simulink model "Centralized_Cont"  (R2018a)
settings: Solver=VariableStepAuto  StartTime=0.0  StopTime=5  RelTol=1e-3
values from neighbouring files (symbols this model uses):
  Kd_Cent = zeros(7,7)    [ControlSetup.m]
  Kp_Cent = zeros(7,7)    [ControlSetup.m]
libraries: dspinverses x1
(part 4 of 4)

== matlab function Centralized_Cont/Estimator/Dynamics_e ==
  data: dq2 input; B output; dq3 input; dq4 input; dq5 input; dq6 input; dq7 input; g input; q2 input; q3 input; q4 input; q5 input; q6 input; Bm output; phi output; phim output; G output
function [B,Bm,phi,phim,G] = Dynamics_e(dq2,dq3,dq4,dq5,dq6,dq7,g,q2,q3,q4,q5,q6)
%#codegen

%    This function was generated by the Symbolic Math Toolbox version 8.1.
%    29-May-2020 11:22:38

t2 = cos(q2);
t3 = sin(q2);
t4 = sin(q5);
t5 = cos(q3);
t6 = cos(q4);
t7 = sin(q3);
t8 = sin(q4);
t9 = cos(q5);
t10 = cos(q6);
t11 = sin(q6);
t12 = t3.*4.525398e-2;
t13 = t3.*t4.*t11.*1.279539e-2;
t14 = t2.*t5.*t8.*1.27482732;
t15 = t2.*t6.*t7.*1.27482732;
t16 = t2.*t7.*t8.*2.136096e-1;
t17 = t2.*t4.*t5.*t6.*1.612305e-2;
t18 = t2.*t5.*t8.*t10.*1.279539e-2;
t19 = t2.*t6.*t7.*t10.*1.279539e-2;
t20 = t2.*t7.*t8.*t9.*4.1238e-4;
t21 = t2.*t5.*t6.*t9.*t11.*1.279539e-2;
t22 = t2.*(-5.811597e-1)+t12+t13+t14+t15+t16+t17+t18+t19+t20+t21-t2.*t5.*4.3309791-t3.*t4.*4.1238e-4-t2.*t7.*5.866623e-2-t3.*t9.*1.612305e-2-t2.*t5.*t6.*2.136096e-1-t2.*t4.*t7.*t8.*1.612305e-2-t2.*t5.*t6.*t9.*4.1238e-4-t2.*t7.*t8.*t9.*t11.*1.279539e-2;
t23 = t5.^2;
t24 = t6.^2;
t25 = t10.^2;
t26 = t9.^2;
t27 = t5.*t8.*1.484568e-6;
t28 = t6.*t7.*1.484568e-6;
t29 = t4.*t7.*t8.*9.5218542e-5;
t30 = t7.*t8.*t9.*4.194107562e-3;
t31 = t5.*t8.*t11.*t26.*4.2919632e-5;
t32 = t6.*t7.*t11.*t26.*4.2919632e-5;
t33 = t4.*t5.*t8.*t9.*2.159275886e-3;
t34 = t4.*t6.*t7.*t9.*2.159275886e-3;
t35 = t4.*t5.*t6.*t11.*4.67031735e-3;
t36 = t7.*t8.*t9.*t10.*2.1459816e-5;
t37 = t4.*t5.*t8.*t11.*4.4783865e-4;
t38 = t4.*t6.*t7.*t11.*4.4783865e-4;
t39 = t4.*t5.*t8.*t9.*t25.*7.96554327e-4;
t40 = t4.*t6.*t7.*t9.*t25.*7.96554327e-4;
t41 = t4.*t5.*t6.*t10.*t11.*7.96554327e-4;
t42 = t5.*6.880448217896662e19;
t43 = t7.*5.079426005445158e21;
t44 = t7.*t8.*1.495133292529617e21;
t45 = t4.*t5.*t8.*1.890931301356143e19;
t46 = t4.*t6.*t7.*1.890931301356143e19;
t47 = t7.*t8.*t10.*1.5006592092724e19;
t48 = t5.*t8.*t9.*t11.*1.5006592092724e19;
t49 = t6.*t7.*t9.*t11.*1.5006592092724e19;
t50 = t42-t43+t44+t45+t46+t47+t48+t49-t5.*t6.*1.495133292529617e21-t5.*t8.*2.505239882715523e20-t6.*t7.*2.505239882715523e20-t5.*t6.*t10.*1.5006592092724e19-t5.*t8.*t9.*4.836443787330847e17-t6.*t7.*t9.*4.836443787330847e17;
t51 = t7.*1.121030218e-2;
t52 = t4.*t7.*t11.*4.03054785e-3;
t68 = t5.*t8.*t26.*2.969136e-6;
t69 = t6.*t7.*t26.*2.969136e-6;
t70 = t5.*t6.*t9.*4.194107562e-3;
t71 = t4.*t5.*t6.*9.5218542e-5;
t72 = t5.*t8.*t9.*5.6430675e-4;
t73 = t6.*t7.*t9.*5.6430675e-4;
t74 = t4.*t5.*t8.*1.44333e-5;
t75 = t4.*t6.*t7.*1.44333e-5;
t76 = t5.*t8.*t11.*2.1459816e-5;
t77 = t6.*t7.*t11.*2.1459816e-5;
t78 = t5.*t6.*t9.*t10.*2.1459816e-5;
t79 = t4.*t7.*t8.*t11.*4.67031735e-3;
t80 = t4.*t7.*t8.*t10.*t11.*7.96554327e-4;
t53 = t5.*(-3.40264134e-4)+t27+t28+t29+t30+t31+t32+t33+t34+t35+t36+t37+t38+t39+t40+t41+t51+t52-t68-t69-t70-t71-t72-t73-t74-t75-t76-t77-t78-t79-t80-t4.*t7.*1.298997e-4-t7.*t9.*5.07876075e-3;
t54 = t9.*2.88666e-5;
t55 = q5.*2.0;
t56 = sin(t55);
t57 = t10.*9.3406347e-3;
t58 = t25.*7.96554327e-4;
t59 = t4.*t9.*t11.*4.2919632e-5;
t60 = t5.*t6.*1.4164748e7;
t61 = t5.*t8.*2.37344e6;
t62 = t6.*t7.*2.37344e6;
t63 = t5.*t6.*t10.*1.42171e5;
t64 = t5.*t8.*t9.*4.582e3;
t65 = t6.*t7.*t9.*4.582e3;
t66 = t60+t61+t62+t63+t64+t65-t7.*t8.*1.4164748e7-t4.*t5.*t8.*1.79145e5-t4.*t6.*t7.*1.79145e5-t7.*t8.*t10.*1.42171e5-t5.*t8.*t9.*t11.*1.42171e5-t6.*t7.*t9.*t11.*1.42171e5;
t67 = t3.*t66.*9.0e-8;
t81 = t6.*6.7287024e-2;
t82 = t6.*t9.*1.298997e-4;
t84 = t56.*1.484568e-6;
t85 = t4.*1.1286135e-3;
t86 = t9.*t11.*8.956773e-4;
t87 = t26.*2.159275886e-3;
t88 = t25.*t26.*7.96554327e-4;
t83 = t8.*(-4.015706058e-1)+t54+t57+t58+t59+t81+t82-t84-t85-t86-t87-t88-t4.*t6.*5.07876075e-3-t8.*t10.*4.03054785e-3-t6.*t9.*t11.*4.03054785e-3+3.67536334659e-1;
t89 = t9.*4.194107562e-3;
t90 = t4.*9.5218542e-5;
t91 = t9.*t10.*2.1459816e-5;
t92 = t9.*1.201554327e-3;
t93 = t9.*t10.*4.67031735e-3;
t94 = t4.*t11.*2.1459816e-5;
t95 = t4.*t11.*5.0e-6;
t96 = t2.*t9.*4.1238e-4;
t97 = t3.*t5.*t6.*t9.*1.612305e-2;
t98 = t3.*t4.*t5.*t6.*4.1238e-4;
t99 = t3.*t4.*t7.*t8.*t11.*1.279539e-2;
t100 = t96+t97+t98+t99-t2.*t4.*1.612305e-2-t2.*t9.*t11.*1.279539e-2-t3.*t4.*t7.*t8.*4.1238e-4-t3.*t7.*t8.*t9.*1.612305e-2-t3.*t4.*t5.*t6.*t11.*1.279539e-2;
t101 = t4.*4.0307625e-4;
t102 = t4.*t5.*5.07876075e-3;
t103 = t9.*t11.*3.1988475e-4;
t104 = t7.*t8.*1.0957467016e-2;
t105 = t5.*t6.*t25.*7.96554327e-4;
t106 = t4.*t5.*t6.*5.6430675e-4;
t107 = t5.*t8.*t9.*9.5218542e-5;
t108 = t6.*t7.*t9.*9.5218542e-5;
t109 = t5.*t9.*t11.*4.03054785e-3;
t110 = t7.*t8.*t9.*1.44333e-5;
t111 = t5.*t6.*t9.*t11.*4.4783865e-4;
t112 = t9.*(-1.03095e-5)+t101+t102+t103+t104+t105+t106+t107+t108+t109+t110+t111-t5.*t6.*1.0957467016e-2-t5.*t9.*1.298997e-4-t4.*t5.*t8.*4.194107562e-3-t4.*t6.*t7.*4.194107562e-3-t4.*t7.*t8.*5.6430675e-4-t5.*t6.*t9.*1.44333e-5-t7.*t8.*t25.*7.96554327e-4-t4.*t5.*t8.*t10.*2.1459816e-5-t4.*t6.*t7.*t10.*2.1459816e-5-t5.*t8.*t9.*t11.*4.67031735e-3-t6.*t7.*t9.*t11.*4.67031735e-3-t7.*t8.*t9.*t11.*4.4783865e-4-t5.*t8.*t9.*t10.*t11.*7.96554327e-4-t6.*t7.*t9.*t10.*t11.*7.96554327e-4;
t113 = t4.*t8.*t11.*4.03054785e-3;
t115 = t4.*t11.*4.67031735e-3;
t116 = t4.*t10.*t11.*7.96554327e-4;
t114 = t89+t90+t91+t113-t115-t116-t4.*t8.*1.298997e-4-t8.*t9.*5.07876075e-3;
t117 = t3.*t5.*t6.*t9.*t10.*1.279539e-2;
t118 = t117-t2.*t4.*t10.*1.279539e-2-t3.*t5.*t8.*t11.*1.279539e-2-t3.*t6.*t7.*t11.*1.279539e-2-t3.*t7.*t8.*t9.*t10.*1.279539e-2;
t119 = t4.*t10.*3.1988475e-4;
t120 = t4.*t5.*t10.*4.03054785e-3;
t121 = t7.*t8.*t10.*2.1459816e-5;
t122 = t4.*t5.*t6.*t10.*4.4783865e-4;
t123 = t5.*t8.*t9.*t11.*2.1459816e-5;
t124 = t6.*t7.*t9.*t11.*2.1459816e-5;
t125 = t119+t120+t121+t122+t123+t124-t4.*t5.*t8.*1.201554327e-3-t4.*t6.*t7.*1.201554327e-3-t5.*t6.*t10.*2.1459816e-5-t4.*t5.*t8.*t10.*4.67031735e-3-t4.*t6.*t7.*t10.*4.67031735e-3-t4.*t7.*t8.*t10.*4.4783865e-4;
t127 = t11.*4.4783865e-4;
t126 = t92+t93+t94-t127-t6.*t11.*4.03054785e-3-t8.*t9.*t10.*4.03054785e-3;
t128 = t10.*2.1459816e-5;
t129 = q3+q4;
t130 = t10.*5.0e-6;
t131 = q4.*2.0;
t132 = t11.^2;
t133 = t4.*t10.*(2.1e1./1.0e3);
t134 = t9.*t10.*t11.*(2.1e1./1.0e3);
t135 = t133+t134;
t136 = t4.^2;
t140 = t4.*t11;
t137 = t9-t140;
t138 = sin(t129);
t139 = cos(t129);
t141 = dq2.^2;
t142 = dq5.^2;
t143 = dq3.^2;
t144 = dq4.^2;
t145 = dq6.^2;
t146 = q3.*2.0;
t147 = sin(t146);
t148 = cos(t55);
t149 = cos(t146);
t150 = cos(t131);
t151 = sin(t131);
B = reshape([7.8426e1,t22,t3.*t50.*(-8.526512829121202e-22),t67,t100,t118,0.0,t22,t4.*(-1.1286135e-3)+t5.*2.16548955e-1+t7.*2.9333115e-3+t23.*1.610619881558+t24.*3.25881982477e-1-t25.*7.96554327e-4+t54+t147.*5.438968859e-2+t151.*4.520441246e-2+t5.*t6.*1.068048e-2-t5.*t8.*6.3741366e-2-t6.*t7.*6.3741366e-2-t7.*t8.*1.068048e-2-t9.*t11.*8.956773e-4+t4.*t23.*1.1286135e-3+t4.*t24.*1.1286135e-3+t6.*t23.*1.34574048e-1-t8.*t23.*8.031412116e-1-t9.*t23.*2.88666e-5-t9.*t24.*2.88666e-5+t10.*t23.*9.3406347e-3+t10.*t24.*9.3406347e-3-t23.*t24.*6.51763964954e-1+t23.*t25.*7.96554327e-4+t23.*t26.*2.159275886e-3+t24.*t25.*7.96554327e-4+t24.*t26.*2.159275886e-3-t4.*t5.*t6.*8.061525e-4-t4.*t5.*t7.*8.388215124e-3-t4.*t6.*t8.*8.388215124e-3-t5.*t6.*t7.*8.031412116e-1+t4.*t7.*t8.*8.061525e-4+t5.*t6.*t9.*2.0619e-5-t5.*t7.*t8.*1.34574048e-1+t5.*t7.*t9.*1.90437084e-4+t5.*t7.*t10.*8.956773e-4-t5.*t8.*t10.*6.397695e-4-t6.*t7.*t10.*6.397695e-4+t6.*t8.*t9.*1.90437084e-4+t6.*t8.*t10.*8.956773e-4-t7.*t8.*t9.*2.0619e-5-t4.*t6.*t23.*1.01575215e-2+t4.*t9.*t23.*2.969136e-6-t5.*t7.*t24.*1.8081764984e-1+t4.*t9.*t24.*2.969136e-6-t6.*t8.*t23.*1.8081764984e-1+t6.*t9.*t23.*2.597994e-4-t8.*t10.*t23.*8.0610957e-3+t9.*t11.*t23.*8.956773e-4+t9.*t11.*t24.*8.956773e-4-t4.*t23.*t24.*2.257227e-3+t9.*t23.*t24.*5.77332e-5-t10.*t23.*t24.*1.86812694e-2-t23.*t24.*t25.*1.593108654e-3-t23.*t24.*t26.*4.318551772e-3+t23.*t25.*t26.*7.96554327e-4+t24.*t25.*t26.*7.96554327e-4+t4.*t5.*t7.*t8.*1.01575215e-2-t4.*t5.*t7.*t10.*4.2919632e-5+t5.*t6.*t7.*t8.*6.51763964954e-1-t4.*t6.*t8.*t10.*4.2919632e-5-t5.*t6.*t7.*t10.*8.0610957e-3-t5.*t7.*t8.*t9.*2.597994e-4-t5.*t6.*t9.*t11.*6.397695e-4-t5.*t7.*t9.*t11.*9.3406347e-3-t6.*t8.*t9.*t11.*9.3406347e-3+t7.*t8.*t9.*t11.*6.397695e-4+t4.*t5.*t7.*t24.*1.6776430248e-2+t4.*t6.*t8.*t23.*1.6776430248e-2-t5.*t7.*t9.*t24.*3.80874168e-4-t5.*t7.*t10.*t24.*1.7913546e-3-t6.*t8.*t9.*t23.*3.80874168e-4-t4.*t9.*t11.*t23.*4.2919632e-5-t6.*t8.*t10.*t23.*1.7913546e-3-t4.*t9.*t11.*t24.*4.2919632e-5-t6.*t9.*t11.*t23.*8.0610957e-3-t4.*t9.*t23.*t24.*5.938272e-6-t9.*t11.*t23.*t24.*1.7913546e-3-t23.*t24.*t25.*t26.*1.593108654e-3+t4.*t5.*t6.*t7.*t8.*2.257227e-3-t5.*t6.*t7.*t8.*t9.*5.77332e-5+t5.*t6.*t7.*t8.*t10.*1.86812694e-2+t5.*t7.*t8.*t9.*t11.*8.0610957e-3-t5.*t7.*t9.*t10.*t11.*1.593108654e-3-t6.*t8.*t9.*t10.*t11.*1.593108654e-3+t4.*t5.*t7.*t10.*t24.*8.5839264e-5+t4.*t6.*t8.*t10.*t23.*8.5839264e-5+t5.*t6.*t7.*t8.*t25.*1.593108654e-3+t5.*t6.*t7.*t8.*t26.*4.318551772e-3+t5.*t7.*t9.*t11.*t24.*1.86812694e-2+t6.*t8.*t9.*t11.*t23.*1.86812694e-2+t4.*t9.*t11.*t23.*t24.*8.5839264e-5+t4.*t5.*t6.*t7.*t8.*t9.*5.938272e-6+t5.*t6.*t7.*t8.*t9.*t11.*1.7913546e-3+t5.*t7.*t9.*t10.*t11.*t24.*3.186217308e-3+t6.*t8.*t9.*t10.*t11.*t23.*3.186217308e-3+t5.*t6.*t7.*t8.*t25.*t26.*1.593108654e-3-t4.*t5.*t6.*t7.*t8.*t9.*t11.*8.5839264e-5+2.03088070899e-1,t53,t27+t28+t29+t30+t31+t32+t33+t34+t35+t36+t37+t38+t39+t40+t41-t68-t69-t70-t71-t72-t73-t74-t75-t76-t77-t78-t79-t80,t112,t125,t10.*t139.*(-5.0e-6)+t9.*t11.*t138.*5.0e-6,t3.*t50.*(-8.526512829121202e-22),t53,t4.*(-1.1286135e-3)+t6.*1.34574048e-1-t8.*8.031412116e-1-t26.*2.159275886e-3+t54-t56.*1.484568e-6+t57+t58+t59-t4.*t6.*1.01575215e-2+t6.*t9.*2.597994e-4-t8.*t10.*8.0610957e-3-t9.*t11.*8.956773e-4-t25.*t26.*7.96554327e-4-t6.*t9.*t11.*8.0610957e-3+1.690796095778,t83,t114,t126,t95,t67,t27+t28+t29+t30+t31+t32+t33+t34+t35+t36+t37+t38+t39+t40+t41-t4.*t5.*t6.*9.5218542e-5-t4.*t5.*t8.*1.44333e-5-t4.*t6.*t7.*1.44333e-5-t5.*t6.*t9.*4.194107562e-3-t5.*t8.*t9.*5.6430675e-4-t6.*t7.*t9.*5.6430675e-4-t5.*t8.*t11.*2.1459816e-5-t6.*t7.*t11.*2.1459816e-5-t5.*t8.*t26.*2.969136e-6-t6.*t7.*t26.*2.969136e-6-t4.*t7.*t8.*t11.*4.67031735e-3-t5.*t6.*t9.*t10.*2.1459816e-5-t4.*t7.*t8.*t10.*t11.*7.96554327e-4,t83,t54+t57+t58+t59-t84-t85-t86-t87-t88+3.67536334659e-1,t89+t90+t91-t115-t116,t92+t93+t94-t127,t95,t100,t112,t114,t89+t90+t91-t4.*t11.*4.67031735e-3-t4.*t10.*t11.*7.96554327e-4,t132.*7.96554327e-4+1.0160912689e-2,t128,t130,t118,t125,t126,t11.*(-4.4783865e-4)+t92+t93+t94,t128,1.201554327e-3,0.0,0.0,-t5.*(t6.*t10.*5.0e-6-t8.*t9.*t11.*5.0e-6)+t7.*(t8.*t10.*5.0e-6+t6.*t9.*t11.*5.0e-6),t95,t95,t130,0.0,5.0e-6],[7,7]);
if nargout > 1
    Bm = reshape([2.1e1./1.0e1,0.0,0.0,0.0,0.0,0.0,0.0,0.0,2.1e1./1.0e1,t2.*(-2.1e1./1.0e3),0.0,t8.*t138.*(2.1e1./1.0e3),t9.*t139.*(2.1e1./1.0e3)-t56.*t138.*1.05e-2,t11.*(t11.*t139.*(2.1e1./1.0e3)+t9.*t10.*t138.*(2.1e1./1.0e3))+t4.*t10.*t138.*(2.1e1./1.0e3),0.0,t2.*(-2.1e1./1.0e3),2.1e1./1.0e1,2.1e1./1.0e3,t6.*(-2.1e1./1.0e3),t136.*(-2.1e1./1.0e3),t10.*t137.*(-2.1e1./1.0e3),0.0,0.0,2.1e1./1.0e3,2.1e1./1.0e1,t6.*(-2.1e1./1.0e3),t136.*(-2.1e1./1.0e3),t10.*t137.*(-2.1e1./1.0e3),0.0,t5.*1.05e-2-cos(q3+t131).*1.05e-2,t6.*(-2.1e1./1.0e3),t6.*(-2.1e1./1.0e3),2.1e1./1.0e1,t9.*(-2.1e1./1.0e3),t132.*(-2.1e1./1.0e3),0.0,t5.*(t6.*t9.*(2.1e1./1.0e3)-t4.*t8.*t9.*(2.1e1./1.0e3))-t7.*(t8.*t9.*(2.1e1./1.0e3)+t4.*t6.*t9.*(2.1e1./1.0e3)),t136.*(-2.1e1./1.0e3),t136.*(-2.1e1./1.0e3),t9.*(-2.1e1./1.0e3),2.1e1./1.0e1,t10.*(-2.1e1./1.0e3),0.0,t5.*(t6.*t132.*(2.1e1./1.0e3)+t8.*t135)-t7.*(t8.*t132.*(2.1e1./1.0e3)-t6.*t135),t10.*t137.*(-2.1e1./1.0e3),t10.*t137.*(-2.1e1./1.0e3),t132.*(-2.1e1./1.0e3),t10.*(-2.1e1./1.0e3),2.1e1./1.0e1],[7,7]);
end
if nargout > 2
    t152 = q6.*2.0;
    t153 = sin(t152);
    t154 = cos(t152);
    t155 = t9.*t142.*9.5218542e-5;
    t156 = t5.*t6.*t141.*3.1870683e-2;
    t157 = t5.*t8.*t141.*5.34024e-3;
    t158 = t6.*t7.*t141.*5.34024e-3;
    t159 = t4.*t10.*t145.*2.1459816e-5;
    t160 = t5.*t6.*t10.*t141.*3.1988475e-4;
    t161 = t5.*t8.*t9.*t141.*1.03095e-5;
    t162 = t6.*t7.*t9.*t141.*1.03095e-5;
    t163 = dq5.*dq7.*t9.*t11.*5.0e-6;
    t164 = dq6.*dq7.*t4.*t10.*5.0e-6;
    t165 = dq3.*dq5.*t4.*t11.*8.956773e-4;
    t166 = dq4.*dq5.*t4.*t11.*8.956773e-4;
    t167 = dq2.*dq5.*t4.*t5.*t6.*8.388215124e-3;
    t168 = dq2.*dq5.*t4.*t5.*t8.*1.1286135e-3;
    t169 = dq2.*dq5.*t4.*t6.*t7.*1.1286135e-3;
    t170 = dq2.*dq5.*t7.*t8.*t9.*1.90437084e-4;
    t171 = dq2.*dq5.*t5.*t6.*t9.*t11.*9.3406347e-3;
    t172 = dq2.*dq5.*t4.*t5.*t6.*t10.*4.2919632e-5;
    t173 = dq2.*dq6.*t4.*t5.*t6.*t10.*9.3406347e-3;
    t174 = dq2.*dq5.*t5.*t8.*t9.*t11.*8.956773e-4;
    t175 = dq2.*dq5.*t6.*t7.*t9.*t11.*8.956773e-4;
    t176 = dq2.*dq6.*t4.*t5.*t8.*t10.*8.956773e-4;
    t177 = dq2.*dq6.*t4.*t6.*t7.*t10.*8.956773e-4;
    t178 = dq2.*dq7.*t7.*t8.*t9.*t11.*5.0e-6;
    phi = [t2.*t141.*4.525398e-2+t3.*t141.*5.811597e-1-t2.*t4.*t141.*4.1238e-4-t2.*t4.*t142.*4.1238e-4+t3.*t5.*t141.*4.3309791+t3.*t5.*t143.*4.3309791+t3.*t7.*t141.*5.866623e-2-t2.*t9.*t141.*1.612305e-2-t2.*t9.*t142.*1.612305e-2+t3.*t7.*t143.*5.866623e-2-dq2.*dq3.*t2.*t5.*1.1733246e-1+dq2.*dq3.*t2.*t7.*8.6619582+dq2.*dq5.*t3.*t4.*3.22461e-2-dq2.*dq5.*t3.*t9.*8.2476e-4+t3.*t5.*t6.*t141.*2.136096e-1+t3.*t5.*t6.*t143.*2.136096e-1-t3.*t5.*t8.*t141.*1.27482732-t3.*t6.*t7.*t141.*1.27482732+t2.*t4.*t11.*t141.*1.279539e-2+t3.*t5.*t6.*t144.*2.136096e-1+t2.*t4.*t11.*t142.*1.279539e-2-t3.*t5.*t8.*t143.*1.27482732-t3.*t6.*t7.*t143.*1.27482732-t3.*t7.*t8.*t141.*2.136096e-1-t3.*t5.*t8.*t144.*1.27482732-t3.*t6.*t7.*t144.*1.27482732-t3.*t7.*t8.*t143.*2.136096e-1+t2.*t4.*t11.*t145.*1.279539e-2-t3.*t7.*t8.*t144.*2.136096e-1+dq2.*dq3.*t2.*t5.*t6.*2.54965464+dq2.*dq4.*t2.*t5.*t6.*2.54965464+dq2.*dq3.*t2.*t5.*t8.*4.272192e-1+dq2.*dq3.*t2.*t6.*t7.*4.272192e-1+dq2.*dq4.*t2.*t5.*t8.*4.272192e-1+dq2.*dq4.*t2.*t6.*t7.*4.272192e-1+dq3.*dq4.*t3.*t5.*t6.*4.272192e-1-dq2.*dq3.*t2.*t7.*t8.*2.54965464-dq2.*dq4.*t2.*t7.*t8.*2.54965464-dq3.*dq4.*t3.*t5.*t8.*2.54965464-dq3.*dq4.*t3.*t6.*t7.*2.54965464+dq2.*dq6.*t3.*t4.*t10.*2.559078e-2-dq3.*dq4.*t3.*t7.*t8.*4.272192e-1+dq2.*dq5.*t3.*t9.*t11.*2.559078e-2-dq5.*dq6.*t2.*t9.*t10.*2.559078e-2-t3.*t4.*t5.*t6.*t141.*1.612305e-2-t3.*t4.*t5.*t6.*t142.*1.612305e-2-t3.*t4.*t5.*t6.*t143.*1.612305e-2-t3.*t4.*t5.*t6.*t144.*1.612305e-2+t3.*t4.*t7.*t8.*t141.*1.612305e-2+t3.*t4.*t7.*t8.*t142.*1.612305e-2+t3.*t5.*t6.*t9.*t141.*4.1238e-4+t3.*t4.*t7.*t8.*t143.*1.612305e-2+t3.*t5.*t6.*t9.*t142.*4.1238e-4+t3.*t4.*t7.*t8.*t144.*1.612305e-2+t3.*t5.*t6.*t9.*t143.*4.1238e-4+t3.*t5.*t6.*t9.*t144.*4.1238e-4-t3.*t5.*t8.*t10.*t141.*1.279539e-2-t3.*t6.*t7.*t10.*t141.*1.279539e-2-t3.*t7.*t8.*t9.*t141.*4.1238e-4-t3.*t5.*t8.*t10.*t143.*1.279539e-2-t3.*t6.*t7.*t10.*t143.*1.279539e-2-t3.*t7.*t8.*t9.*t142.*4.1238e-4-t3.*t5.*t8.*t10.*t144.*1.279539e-2-t3.*t6.*t7.*t10.*t144.*1.279539e-2-t3.*t7.*t8.*t9.*t143.*4.1238e-4-t3.*t5.*t8.*t10.*t145.*1.279539e-2-t3.*t6.*t7.*t10.*t145.*1.279539e-2-t3.*t7.*t8.*t9.*t144.*4.1238e-4-t3.*t5.*t6.*t9.*t11.*t141.*1.279539e-2-t3.*t5.*t6.*t9.*t11.*t142.*1.279539e-2-t3.*t5.*t6.*t9.*t11.*t143.*1.279539e-2-t3.*t5.*t6.*t9.*t11.*t144.*1.279539e-2-t3.*t5.*t6.*t9.*t11.*t145.*1.279539e-2+t3.*t7.*t8.*t9.*t11.*t141.*1.279539e-2+t3.*t7.*t8.*t9.*t11.*t142.*1.279539e-2+t3.*t7.*t8.*t9.*t11.*t143.*1.279539e-2+t3.*t7.*t8.*t9.*t11.*t144.*1.279539e-2+t3.*t7.*t8.*t9.*t11.*t145.*1.279539e-2-dq2.*dq3.*t2.*t4.*t5.*t8.*3.22461e-2-dq2.*dq3.*t2.*t4.*t6.*t7.*3.22461e-2+dq2.*dq5.*t2.*t4.*t5.*t6.*8.2476e-4-dq2.*dq4.*t2.*t4.*t5.*t8.*3.22461e-2-dq2.*dq4.*t2.*t4.*t6.*t7.*3.22461e-2-dq3.*dq4.*t3.*t4.*t5.*t6.*3.22461e-2+dq2.*dq3.*t2.*t5.*t6.*t10.*2.559078e-2-dq2.*dq5.*t2.*t4.*t7.*t8.*8.2476e-4-dq3.*dq5.*t3.*t4.*t5.*t8.*8.2476e-4-dq3.*dq5.*t3.*t4.*t6.*t7.*8.2476e-4+dq2.*dq3.*t2.*t5.*t8.*t9.*8.2476e-4+dq2.*dq3.*t2.*t6.*t7.*t9.*8.2476e-4+dq2.*dq4.*t2.*t5.*t6.*t10.*2.559078e-2+dq2.*dq5.*t2.*t5.*t6.*t9.*3.22461e-2+dq3.*dq4.*t3.*t4.*t7.*t8.*3.22461e-2-dq4.*dq5.*t3.*t4.*t5.*t8.*8.2476e-4-dq4.*dq5.*t3.*t4.*t6.*t7.*8.2476e-4+dq2.*dq4.*t2.*t5.*t8.*t9.*8.2476e-4+dq2.*dq4.*t2.*t6.*t7.*t9.*8.2476e-4+dq3.*dq4.*t3.*t5.*t6.*t9.*8.2476e-4-dq2.*dq3.*t2.*t7.*t8.*t10.*2.559078e-2-dq2.*dq4.*t2.*t7.*t8.*t10.*2.559078e-2-dq2.*dq5.*t2.*t7.*t8.*t9.*3.22461e-2-dq3.*dq4.*t3.*t5.*t8.*t10.*2.559078e-2-dq3.*dq4.*t3.*t6.*t7.*t10.*2.559078e-2-dq3.*dq5.*t3.*t5.*t8.*t9.*3.22461e-2-dq3.*dq5.*t3.*t6.*t7.*t9.*3.22461e-2-dq2.*dq6.*t2.*t5.*t8.*t11.*2.559078e-2-dq2.*dq6.*t2.*t6.*t7.*t11.*2.559078e-2-dq3.*dq4.*t3.*t7.*t8.*t9.*8.2476e-4-dq3.*dq6.*t3.*t5.*t6.*t11.*2.559078e-2-dq4.*dq5.*t3.*t5.*t8.*t9.*3.22461e-2-dq4.*dq5.*t3.*t6.*t7.*t9.*3.22461e-2-dq4.*dq6.*t3.*t5.*t6.*t11.*2.559078e-2+dq3.*dq6.*t3.*t7.*t8.*t11.*2.559078e-2+dq4.*dq6.*t3.*t7.*t8.*t11.*2.559078e-2-dq2.*dq5.*t2.*t4.*t5.*t6.*t11.*2.559078e-2+dq2.*dq5.*t2.*t4.*t7.*t8.*t11.*2.559078e-2+dq3.*dq5.*t3.*t4.*t5.*t8.*t11.*2.559078e-2+dq3.*dq5.*t3.*t4.*t6.*t7.*t11.*2.559078e-2-dq5.*dq6.*t3.*t4.*t5.*t6.*t10.*2.559078e-2-dq2.*dq3.*t2.*t5.*t8.*t9.*t11.*2.559078e-2-dq2.*dq3.*t2.*t6.*t7.*t9.*t11.*2.559078e-2+dq2.*dq6.*t2.*t5.*t6.*t9.*t10.*2.559078e-2+dq4.*dq5.*t3.*t4.*t5.*t8.*t11.*2.559078e-2+dq4.*dq5.*t3.*t4.*t6.*t7.*t11.*2.559078e-2-dq2.*dq4.*t2.*t5.*t8.*t9.*t11.*2.559078e-2-dq2.*dq4.*t2.*t6.*t7.*t9.*t11.*2.559078e-2-dq3.*dq4.*t3.*t5.*t6.*t9.*t11.*2.559078e-2+dq5.*dq6.*t3.*t4.*t7.*t8.*t10.*2.559078e-2-dq2.*dq6.*t2.*t7.*t8.*t9.*t10.*2.559078e-2-dq3.*dq6.*t3.*t5.*t8.*t9.*t10.*2.559078e-2-dq3.*dq6.*t3.*t6.*t7.*t9.*t10.*2.559078e-2+dq3.*dq4.*t3.*t7.*t8.*t9.*t11.*2.559078e-2-dq4.*dq6.*t3.*t5.*t8.*t9.*t10.*2.559078e-2-dq4.*dq6.*t3.*t6.*t7.*t9.*t10.*2.559078e-2,t4.*t142.*1.03095e-5+t5.*t143.*1.121030218e-2+t7.*t143.*3.40264134e-4+t9.*t142.*4.0307625e-4+dq2.*dq3.*t5.*2.9333115e-3-dq2.*dq5.*t4.*1.44333e-5-dq2.*dq3.*t7.*2.16548955e-1-dq2.*dq4.*t6.*4.015706058e-1-dq2.*dq4.*t8.*6.7287024e-2-dq2.*dq5.*t9.*5.6430675e-4-dq2.*dq6.*t11.*4.67031735e-3-dq2.*dq5.*t56.*1.27877652475e-3-dq2.*dq3.*t147.*1.284737899081+dq2.*dq3.*t149.*1.837055226e-2+dq2.*dq5.*t148.*1.484568e-6+dq2.*dq6.*t153.*1.9913858175e-4+t4.*t5.*t142.*1.298997e-4-t4.*t5.*t143.*1.298997e-4+t5.*t9.*t142.*5.07876075e-3-t4.*t11.*t142.*3.1988475e-4-t5.*t9.*t143.*5.07876075e-3-t4.*t11.*t145.*3.1988475e-4-dq2.*dq3.*t5.*t6.*6.3741366e-2-dq2.*dq4.*t5.*t6.*6.3741366e-2-dq2.*dq5.*t4.*t6.*1.298997e-4-dq2.*dq3.*t5.*t8.*1.068048e-2-dq2.*dq3.*t6.*t7.*1.068048e-2+dq2.*dq4.*t4.*t8.*5.07876075e-3-dq2.*dq4.*t5.*t8.*1.068048e-2-dq2.*dq4.*t6.*t7.*1.068048e-2+dq2.*dq3.*t7.*t8.*6.3741366e-2+dq2.*dq4.*t7.*t8.*6.3741366e-2+dq3.*dq5.*t5.*t8.*1.05591898525e-2+dq3.*dq5.*t6.*t7.*1.05591898525e-2-dq2.*dq4.*t6.*t10.*4.03054785e-3+dq2.*dq5.*t4.*t11.*4.4783865e-4-dq2.*dq5.*t6.*t9.*5.07876075e-3+dq4.*dq5.*t5.*t8.*1.05591898525e-2+dq4.*dq5.*t6.*t7.*1.05591898525e-2-dq2.*dq4.*t8.*t9.*1.298997e-4+dq2.*dq6.*t8.*t11.*4.03054785e-3-dq2.*dq6.*t9.*t10.*4.4783865e-4+dq5.*dq6.*t9.*t10.*6.397695e-4-dq2.*dq6.*t10.*t56.*1.0729908e-5-dq2.*dq3.*t6.*t147.*1.34574048e-1-dq2.*dq4.*t6.*t147.*6.7287024e-2-dq2.*dq3.*t6.*t149.*8.031412116e-1+dq2.*dq3.*t8.*t147.*8.031412116e-1-dq2.*dq4.*t6.*t149.*4.015706058e-1+dq2.*dq4.*t8.*t147.*4.015706058e-1-dq2.*dq3.*t8.*t149.*1.34574048e-1-dq2.*dq4.*t8.*t149.*6.7287024e-2-dq2.*dq5.*t11.*t148.*2.1459816e-5-dq2.*dq5.*t56.*t154.*1.9913858175e-4+dq2.*dq3.*t147.*t150.*3.2755903616525e-1+dq2.*dq3.*t147.*t151.*9.040882492e-2+dq2.*dq4.*t147.*t150.*3.2755903616525e-1-dq2.*dq3.*t149.*t150.*9.040882492e-2+dq2.*dq4.*t147.*t151.*9.040882492e-2+dq2.*dq3.*t149.*t151.*3.2755903616525e-1-dq2.*dq4.*t149.*t150.*9.040882492e-2+dq2.*dq4.*t149.*t151.*3.2755903616525e-1-dq2.*dq6.*t148.*t153.*1.9913858175e-4+t4.*t5.*t6.*t142.*1.44333e-5-t4.*t5.*t6.*t143.*1.44333e-5-t4.*t5.*t6.*t144.*1.44333e-5-t4.*t5.*t8.*t142.*9.5218542e-5-t4.*t6.*t7.*t142.*9.5218542e-5+t4.*t5.*t8.*t143.*9.5218542e-5+t4.*t6.*t7.*t143.*9.5218542e-5+t4.*t5.*t8.*t144.*9.5218542e-5+t4.*t6.*t7.*t144.*9.5218542e-5-t4.*t7.*t8.*t142.*1.44333e-5-t4.*t5.*t11.*t142.*4.03054785e-3+t4.*t7.*t8.*t143.*1.44333e-5+t5.*t6.*t9.*t142.*5.6430675e-4+t4.*t5.*t11.*t143.*4.03054785e-3+t4.*t7.*t8.*t144.*1.44333e-5-t5.*t6.*t9.*t143.*5.6430675e-4-t5.*t6.*t9.*t144.*5.6430675e-4-t5.*t8.*t9.*t142.*4.194107562e-3-t6.*t7.*t9.*t142.*4.194107562e-3-t4.*t5.*t11.*t145.*4.03054785e-3+t5.*t8.*t9.*t143.*4.194107562e-3+t6.*t7.*t9.*t143.*4.194107562e-3+t5.*t8.*t9.*t144.*4.194107562e-3+t6.*t7.*t9.*t144.*4.194107562e-3-t7.*t8.*t9.*t142.*5.6430675e-4+t5.*t6.*t11.*t145.*2.1459816e-5+t7.*t8.*t9.*t143.*5.6430675e-4+t7.*t8.*t9.*t144.*5.6430675e-4-t7.*t8.*t11.*t145.*2.1459816e-5+t5.*t6.*t56.*t143.*1.27877652475e-3+t5.*t6.*t56.*t144.*1.27877652475e-3-t7.*t8.*t56.*t143.*1.27877652475e-3-t7.*t8.*t56.*t144.*1.27877652475e-3-t5.*t6.*t143.*t148.*1.484568e-6-t5.*t6.*t144.*t148.*1.484568e-6+t7.*t8.*t143.*t148.*1.484568e-6+t7.*t8.*t144.*t148.*1.484568e-6+dq2.*dq3.*t4.*t5.*t8.*8.061525e-4+dq2.*dq3.*t4.*t6.*t7.*8.061525e-4-dq2.*dq5.*t4.*t5.*t6.*2.0619e-5-dq3.*dq4.*t4.*t5.*t6.*2.88666e-5+dq2.*dq4.*t4.*t5.*t8.*8.061525e-4+dq2.*dq4.*t4.*t6.*t7.*8.061525e-4+dq3.*dq4.*t4.*t5.*t8.*1.90437084e-4+dq3.*dq4.*t4.*t6.*t7.*1.90437084e-4-dq3.*dq6.*t4.*t5.*t6.*1.201554327e-3-dq4.*dq6.*t4.*t5.*t6.*1.201554327e-3-dq2.*dq3.*t5.*t6.*t10.*6.397695e-4+dq2.*dq5.*t4.*t7.*t8.*2.0619e-5+dq3.*dq4.*t4.*t7.*t8.*2.88666e-5-dq2.*dq3.*t5.*t8.*t9.*2.0619e-5-dq2.*dq3.*t6.*t7.*t9.*2.0619e-5-dq2.*dq4.*t5.*t6.*t10.*6.397695e-4-dq2.*dq5.*t5.*t6.*t9.*8.061525e-4-dq3.*dq4.*t5.*t6.*t9.*1.1286135e-3-dq2.*dq4.*t5.*t8.*t9.*2.0619e-5-dq2.*dq4.*t6.*t7.*t9.*2.0619e-5+dq2.*dq5.*t4.*t6.*t11.*4.03054785e-3+dq3.*dq6.*t4.*t7.*t8.*1.201554327e-3+dq3.*dq4.*t5.*t8.*t9.*8.388215124e-3+dq3.*dq4.*t6.*t7.*t9.*8.388215124e-3+dq4.*dq6.*t4.*t7.*t8.*1.201554327e-3+dq2.*dq3.*t7.*t8.*t10.*6.397695e-4+dq2.*dq4.*t7.*t8.*t10.*6.397695e-4+dq2.*dq5.*t7.*t8.*t9.*8.061525e-4+dq3.*dq4.*t7.*t8.*t9.*1.1286135e-3+dq2.*dq6.*t5.*t8.*t11.*6.397695e-4+dq2.*dq6.*t6.*t7.*t11.*6.397695e-4+dq3.*dq6.*t5.*t8.*t10.*2.1459816e-5+dq3.*dq6.*t6.*t7.*t10.*2.1459816e-5-dq2.*dq6.*t6.*t9.*t10.*4.03054785e-3+dq3.*dq7.*t5.*t8.*t10.*5.0e-6+dq3.*dq7.*t6.*t7.*t10.*5.0e-6+dq4.*dq6.*t5.*t8.*t10.*2.1459816e-5+dq4.*dq6.*t6.*t7.*t10.*2.1459816e-5-dq5.*dq6.*t5.*t8.*t9.*1.201554327e-3-dq5.*dq6.*t6.*t7.*t9.*1.201554327e-3+dq2.*dq4.*t8.*t9.*t11.*4.03054785e-3+dq4.*dq7.*t5.*t8.*t10.*5.0e-6+dq4.*dq7.*t6.*t7.*t10.*5.0e-6+dq5.*dq6.*t5.*t9.*t10.*8.0610957e-3+dq6.*dq7.*t5.*t6.*t11.*5.0e-6-dq6.*dq7.*t7.*t8.*t11.*5.0e-6+dq3.*dq4.*t5.*t6.*t56.*2.5575530495e-3+dq3.*dq5.*t5.*t8.*t56.*2.969136e-6+dq3.*dq5.*t6.*t7.*t56.*2.969136e-6-dq3.*dq4.*t7.*t8.*t56.*2.5575530495e-3+dq4.*dq5.*t5.*t8.*t56.*2.969136e-6+dq4.*dq5.*t6.*t7.*t56.*2.969136e-6+dq2.*dq3.*t4.*t6.*t147.*1.01575215e-2+dq2.*dq4.*t4.*t6.*t147.*5.07876075e-3+dq2.*dq3.*t4.*t8.*t149.*1.01575215e-2-dq2.*dq5.*t4.*t6.*t149.*1.298997e-4+dq2.*dq5.*t4.*t8.*t147.*1.298997e-4-dq3.*dq4.*t5.*t6.*t148.*2.969136e-6-dq2.*dq3.*t6.*t9.*t147.*2.597994e-4+dq2.*dq4.*t4.*t8.*t149.*5.07876075e-3-dq2.*dq4.*t6.*t9.*t147.*1.298997e-4+dq3.*dq5.*t5.*t8.*t148.*2.5575530495e-3+dq3.*dq5.*t6.*t7.*t148.*2.5575530495e-3-dq2.*dq3.*t6.*t10.*t149.*8.0610957e-3+dq2.*dq3.*t8.*t10.*t147.*8.0610957e-3+dq3.*dq4.*t7.*t8.*t148.*2.969136e-6+dq4.*dq5.*t5.*t8.*t148.*2.5575530495e-3+dq4.*dq5.*t6.*t7.*t148.*2.5575530495e-3-dq2.*dq3.*t8.*t9.*t149.*2.597994e-4-dq2.*dq4.*t6.*t10.*t149.*4.03054785e-3+dq2.*dq4.*t8.*t10.*t147.*4.03054785e-3-dq2.*dq5.*t6.*t9.*t149.*5.07876075e-3+dq2.*dq5.*t8.*t9.*t147.*5.07876075e-3-dq2.*dq4.*t8.*t9.*t149.*1.298997e-4+dq2.*dq6.*t6.*t11.*t147.*4.03054785e-3-dq3.*dq5.*t5.*t8.*t154.*3.982771635e-4-dq3.*dq5.*t6.*t7.*t154.*3.982771635e-4-dq5.*dq6.*t5.*t6.*t153.*7.96554327e-4+dq2.*dq6.*t8.*t11.*t149.*4.03054785e-3-dq4.*dq5.*t5.*t8.*t154.*3.982771635e-4-dq4.*dq5.*t6.*t7.*t154.*3.982771635e-4+dq5.*dq6.*t7.*t8.*t153.*7.96554327e-4+dq2.*dq3.*t4.*t147.*t150.*1.1286135e-3-dq2.*dq3.*t4.*t147.*t151.*8.388215124e-3+dq2.*dq4.*t4.*t147.*t150.*1.1286135e-3+dq2.*dq3.*t4.*t149.*t150.*8.388215124e-3-dq2.*dq4.*t4.*t147.*t151.*8.388215124e-3+dq2.*dq5.*t4.*t147.*t150.*9.5218542e-5+dq2.*dq3.*t4.*t149.*t151.*1.1286135e-3+dq2.*dq4.*t4.*t149.*t150.*8.388215124e-3+dq2.*dq5.*t4.*t147.*t151.*1.44333e-5+dq2.*dq4.*t4.*t149.*t151.*1.1286135e-3-dq2.*dq5.*t4.*t149.*t150.*1.44333e-5-dq2.*dq3.*t9.*t147.*t150.*2.88666e-5+dq2.*dq5.*t4.*t149.*t151.*9.5218542e-5+dq2.*dq3.*t9.*t147.*t151.*1.90437084e-4+dq2.*dq3.*t10.*t147.*t150.*9.3406347e-3-dq2.*dq4.*t9.*t147.*t150.*2.88666e-5-dq2.*dq3.*t9.*t149.*t150.*1.90437084e-4+dq2.*dq3.*t10.*t147.*t151.*8.956773e-4+dq2.*dq4.*t9.*t147.*t151.*1.90437084e-4+dq2.*dq4.*t10.*t147.*t150.*9.3406347e-3+dq2.*dq5.*t9.*t147.*t150.*4.194107562e-3-dq2.*dq3.*t9.*t149.*t151.*2.88666e-5-dq2.*dq3.*t10.*t149.*t150.*8.956773e-4-dq2.*dq4.*t9.*t149.*t150.*1.90437084e-4+dq2.*dq4.*t10.*t147.*t151.*8.956773e-4+dq2.*dq5.*t9.*t147.*t151.*5.6430675e-4+dq2.*dq3.*t10.*t149.*t151.*9.3406347e-3-dq2.*dq4.*t9.*t149.*t151.*2.88666e-5-dq2.*dq4.*t10.*t149.*t150.*8.956773e-4-dq2.*dq5.*t9.*t149.*t150.*5.6430675e-4+dq2.*dq4.*t10.*t149.*t151.*9.3406347e-3+dq2.*dq5.*t9.*t149.*t151.*4.194107562e-3+dq2.*dq6.*t11.*t147.*t150.*4.4783865e-4-dq2.*dq6.*t11.*t147.*t151.*4.67031735e-3+dq2.*dq6.*t11.*t149.*t150.*4.67031735e-3+dq2.*dq6.*t11.*t149.*t151.*4.4783865e-4+dq2.*dq3.*t56.*t147.*t150.*1.484568e-6+dq2.*dq4.*t56.*t147.*t150.*1.484568e-6+dq2.*dq3.*t56.*t149.*t151.*1.484568e-6-dq2.*dq5.*t56.*t147.*t151.*1.27877652475e-3+dq2.*dq4.*t56.*t149.*t151.*1.484568e-6+dq2.*dq5.*t56.*t149.*t150.*1.27877652475e-3+dq2.*dq3.*t147.*t148.*t150.*1.27877652475e-3+dq2.*dq4.*t147.*t148.*t150.*1.27877652475e-3+dq2.*dq3.*t148.*t149.*t151.*1.27877652475e-3+dq2.*dq5.*t147.*t148.*t151.*1.484568e-6+dq2.*dq4.*t148.*t149.*t151.*1.27877652475e-3-dq2.*dq5.*t148.*t149.*t150.*1.484568e-6+dq2.*dq3.*t147.*t150.*t154.*5.9741574525e-4+dq2.*dq4.*t147.*t150.*t154.*5.9741574525e-4+dq2.*dq3.*t149.*t151.*t154.*5.9741574525e-4-dq2.*dq6.*t147.*t151.*t153.*5.9741574525e-4+dq2.*dq4.*t149.*t151.*t154.*5.9741574525e-4+dq2.*dq6.*t149.*t150.*t153.*5.9741574525e-4-t4.*t5.*t6.*t11.*t142.*4.4783865e-4+t4.*t5.*t6.*t11.*t143.*4.4783865e-4+t4.*t5.*t6.*t11.*t144.*4.4783865e-4+t4.*t5.*t8.*t11.*t142.*4.67031735e-3+t4.*t6.*t7.*t11.*t142.*4.67031735e-3-t4.*t5.*t6.*t11.*t145.*4.4783865e-4-t4.*t5.*t8.*t11.*t143.*4.67031735e-3-t4.*t6.*t7.*t11.*t143.*4.67031735e-3-t4.*t5.*t8.*t11.*t144.*4.67031735e-3-t4.*t6.*t7.*t11.*t144.*4.67031735e-3+t4.*t7.*t8.*t11.*t142.*4.4783865e-4+t4.*t5.*t8.*t11.*t145.*4.67031735e-3+t4.*t6.*t7.*t11.*t145.*4.67031735e-3-t4.*t7.*t8.*t11.*t143.*4.4783865e-4-t4.*t7.*t8.*t11.*t144.*4.4783865e-4-t5.*t8.*t9.*t10.*t142.*2.1459816e-5-t6.*t7.*t9.*t10.*t142.*2.1459816e-5+t4.*t7.*t8.*t11.*t145.*4.4783865e-4+t5.*t8.*t9.*t10.*t143.*2.1459816e-5+t6.*t7.*t9.*t10.*t143.*2.1459816e-5+t5.*t8.*t9.*t10.*t144.*2.1459816e-5+t6.*t7.*t9.*t10.*t144.*2.1459816e-5+t5.*t8.*t9.*t10.*t145.*2.1459816e-5+t6.*t7.*t9.*t10.*t145.*2.1459816e-5+t4.*t5.*t8.*t142.*t153.*3.982771635e-4+t4.*t6.*t7.*t142.*t153.*3.982771635e-4-t4.*t5.*t8.*t143.*t153.*3.982771635e-4-t4.*t6.*t7.*t143.*t153.*3.982771635e-4+t5.*t6.*t11.*t143.*t148.*2.1459816e-5-t4.*t5.*t8.*t144.*t153.*3.982771635e-4-t4.*t6.*t7.*t144.*t153.*3.982771635e-4+t5.*t6.*t11.*t144.*t148.*2.1459816e-5-t7.*t8.*t11.*t143.*t148.*2.1459816e-5-t7.*t8.*t11.*t144.*t148.*2.1459816e-5+t5.*t6.*t56.*t143.*t154.*1.9913858175e-4+t5.*t6.*t56.*t144.*t154.*1.9913858175e-4-t7.*t8.*t56.*t143.*t154.*1.9913858175e-4-t7.*t8.*t56.*t144.*t154.*1.9913858175e-4+dq2.*dq5.*t4.*t5.*t6.*t11.*6.397695e-4+dq3.*dq4.*t4.*t5.*t6.*t11.*8.956773e-4-dq3.*dq4.*t4.*t5.*t8.*t11.*9.3406347e-3-dq3.*dq4.*t4.*t6.*t7.*t11.*9.3406347e-3-dq2.*dq5.*t4.*t7.*t8.*t11.*6.397695e-4-dq3.*dq4.*t4.*t7.*t8.*t11.*8.956773e-4+dq2.*dq3.*t5.*t8.*t9.*t11.*6.397695e-4+dq2.*dq3.*t6.*t7.*t9.*t11.*6.397695e-4-dq2.*dq6.*t5.*t6.*t9.*t10.*6.397695e-4+dq2.*dq4.*t5.*t8.*t9.*t11.*6.397695e-4+dq2.*dq4.*t6.*t7.*t9.*t11.*6.397695e-4+dq3.*dq4.*t5.*t8.*t9.*t10.*4.2919632e-5+dq3.*dq4.*t6.*t7.*t9.*t10.*4.2919632e-5+dq3.*dq6.*t5.*t6.*t9.*t11.*4.2919632e-5-dq5.*dq7.*t4.*t5.*t8.*t11.*5.0e-6-dq5.*dq7.*t4.*t6.*t7.*t11.*5.0e-6+dq3.*dq7.*t5.*t6.*t9.*t11.*5.0e-6+dq4.*dq6.*t5.*t6.*t9.*t11.*4.2919632e-5+dq5.*dq6.*t5.*t6.*t9.*t10.*8.956773e-4+dq2.*dq6.*t7.*t8.*t9.*t10.*6.397695e-4+dq4.*dq7.*t5.*t6.*t9.*t11.*5.0e-6-dq5.*dq6.*t5.*t8.*t9.*t10.*9.3406347e-3-dq5.*dq6.*t6.*t7.*t9.*t10.*9.3406347e-3-dq3.*dq6.*t7.*t8.*t9.*t11.*4.2919632e-5-dq3.*dq7.*t7.*t8.*t9.*t11.*5.0e-6-dq4.*dq6.*t7.*t8.*t9.*t11.*4.2919632e-5-dq5.*dq6.*t7.*t8.*t9.*t10.*8.956773e-4+dq6.*dq7.*t5.*t8.*t9.*t10.*5.0e-6+dq6.*dq7.*t6.*t7.*t9.*t10.*5.0e-6-dq4.*dq7.*t7.*t8.*t9.*t11.*5.0e-6-dq3.*dq5.*t5.*t8.*t11.*t56.*4.2919632e-5-dq3.*dq5.*t6.*t7.*t11.*t56.*4.2919632e-5-dq4.*dq5.*t5.*t8.*t11.*t56.*4.2919632e-5-dq4.*dq5.*t6.*t7.*t11.*t56.*4.2919632e-5+dq2.*dq5.*t4.*t6.*t11.*t149.*4.03054785e-3-dq2.*dq5.*t4.*t8.*t11.*t147.*4.03054785e-3-dq3.*dq4.*t4.*t5.*t8.*t153.*7.96554327e-4-dq3.*dq4.*t4.*t6.*t7.*t153.*7.96554327e-4+dq3.*dq4.*t5.*t6.*t11.*t148.*4.2919632e-5+dq2.*dq3.*t6.*t9.*t11.*t147.*8.0610957e-3+dq3.*dq6.*t4.*t5.*t6.*t154.*7.96554327e-4+dq2.*dq4.*t6.*t9.*t11.*t147.*4.03054785e-3+dq4.*dq6.*t4.*t5.*t6.*t154.*7.96554327e-4+dq3.*dq6.*t5.*t8.*t10.*t148.*2.1459816e-5+dq3.*dq6.*t6.*t7.*t10.*t148.*2.1459816e-5-dq3.*dq4.*t7.*t8.*t11.*t148.*4.2919632e-5+dq4.*dq6.*t5.*t8.*t10.*t148.*2.1459816e-5+dq4.*dq6.*t6.*t7.*t10.*t148.*2.1459816e-5+dq2.*dq3.*t8.*t9.*t11.*t149.*8.0610957e-3-dq2.*dq6.*t6.*t9.*t10.*t149.*4.03054785e-3+dq2.*dq6.*t8.*t9.*t10.*t147.*4.03054785e-3-dq3.*dq6.*t4.*t7.*t8.*t154.*7.96554327e-4+dq2.*dq4.*t8.*t9.*t11.*t149.*4.03054785e-3-dq4.*dq6.*t4.*t7.*t8.*t154.*7.96554327e-4-dq5.*dq6.*t5.*t8.*t9.*t154.*7.96554327e-4-dq5.*dq6.*t6.*t7.*t9.*t154.*7.96554327e-4+dq3.*dq4.*t5.*t6.*t56.*t154.*3.982771635e-4-dq3.*dq6.*t5.*t8.*t56.*t153.*3.982771635e-4-dq3.*dq6.*t6.*t7.*t56.*t153.*3.982771635e-4-dq3.*dq4.*t7.*t8.*t56.*t154.*3.982771635e-4-dq4.*dq6.*t5.*t8.*t56.*t153.*3.982771635e-4-dq4.*dq6.*t6.*t7.*t56.*t153.*3.982771635e-4-dq2.*dq3.*t4.*t10.*t147.*t151.*4.2919632e-5+dq2.*dq3.*t4.*t10.*t149.*t150.*4.2919632e-5-dq2.*dq4.*t4.*t10.*t147.*t151.*4.2919632e-5+dq2.*dq4.*t4.*t10.*t149.*t150.*4.2919632e-5-dq2.*dq5.*t4.*t11.*t147.*t150.*4.67031735e-3-dq2.*dq5.*t4.*t11.*t147.*t151.*4.4783865e-4-dq2.*dq6.*t4.*t11.*t147.*t150.*2.1459816e-5+dq2.*dq5.*t4.*t11.*t149.*t150.*4.4783865e-4+dq2.*dq3.*t9.*t11.*t147.*t150.*8.956773e-4-dq2.*dq5.*t4.*t11.*t149.*t151.*4.67031735e-3-dq2.*dq3.*t9.*t11.*t147.*t151.*9.3406347e-3+dq2.*dq4.*t9.*t11.*t147.*t150.*8.956773e-4+dq2.*dq5.*t9.*t10.*t147.*t150.*2.1459816e-5-dq2.*dq6.*t4.*t11.*t149.*t151.*2.1459816e-5+dq3.*dq5.*t5.*t8.*t148.*t154.*3.982771635e-4+dq3.*dq5.*t6.*t7.*t148.*t154.*3.982771635e-4+dq2.*dq3.*t9.*t11.*t149.*t150.*9.3406347e-3-dq2.*dq4.*t9.*t11.*t147.*t151.*9.3406347e-3+dq2.*dq6.*t9.*t10.*t147.*t150.*4.67031735e-3+dq4.*dq5.*t5.*t8.*t148.*t154.*3.982771635e-4+dq4.*dq5.*t6.*t7.*t148.*t154.*3.982771635e-4+dq2.*dq3.*t9.*t11.*t149.*t151.*8.956773e-4+dq2.*dq4.*t9.*t11.*t149.*t150.*9.3406347e-3+dq2.*dq6.*t9.*t10.*t147.*t151.*4.4783865e-4+dq2.*dq4.*t9.*t11.*t149.*t151.*8.956773e-4+dq2.*dq5.*t9.*t10.*t149.*t151.*2.1459816e-5-dq2.*dq6.*t9.*t10.*t149.*t150.*4.4783865e-4+dq2.*dq6.*t9.*t10.*t149.*t151.*4.67031735e-3-dq2.*dq3.*t11.*t56.*t147.*t150.*2.1459816e-5-dq2.*dq4.*t11.*t56.*t147.*t150.*2.1459816e-5-dq2.*dq3.*t11.*t56.*t149.*t151.*2.1459816e-5-dq2.*dq6.*t10.*t56.*t147.*t151.*1.0729908e-5-dq2.*dq4.*t11.*t56.*t149.*t151.*2.1459816e-5+dq2.*dq6.*t10.*t56.*t149.*t150.*1.0729908e-5-dq2.*dq5.*t4.*t147.*t150.*t153.*3.982771635e-4-dq2.*dq5.*t4.*t149.*t151.*t153.*3.982771635e-4-dq2.*dq5.*t11.*t147.*t148.*t151.*2.1459816e-5-dq2.*dq3.*t9.*t147.*t151.*t153.*7.96554327e-4+dq2.*dq5.*t11.*t148.*t149.*t150.*2.1459816e-5+dq2.*dq3.*t9.*t149.*t150.*t153.*7.96554327e-4-dq2.*dq4.*t9.*t147.*t151.*t153.*7.96554327e-4+dq2.*dq4.*t9.*t149.*t150.*t153.*7.96554327e-4+dq2.*dq6.*t9.*t147.*t150.*t154.*7.96554327e-4+dq2.*dq6.*t9.*t149.*t151.*t154.*7.96554327e-4-dq2.*dq5.*t56.*t147.*t151.*t154.*1.9913858175e-4+dq2.*dq5.*t56.*t149.*t150.*t154.*1.9913858175e-4+dq2.*dq3.*t147.*t148.*t150.*t154.*1.9913858175e-4+dq2.*dq4.*t147.*t148.*t150.*t154.*1.9913858175e-4+dq2.*dq3.*t148.*t149.*t151.*t154.*1.9913858175e-4-dq2.*dq6.*t147.*t148.*t151.*t153.*1.9913858175e-4+dq2.*dq4.*t148.*t149.*t151.*t154.*1.9913858175e-4+dq2.*dq6.*t148.*t149.*t150.*t153.*1.9913858175e-4,t155+t156+t157+t158+t159+t160+t161+t162+t163+t164+t165+t166+t167+t168+t169+t170+t171+t172+t173+t174+t175+t176+t177+t178-t4.*t142.*4.194107562e-3-t5.*t141.*1.46665575e-3+t7.*t141.*1.082744775e-1-t6.*t144.*4.015706058e-1-t8.*t144.*6.7287024e-2-t10.*t145.*4.4783865e-4+t141.*t147.*6.423689495405e-1-t141.*t149.*9.18527613e-3-dq3.*dq5.*t4.*2.88666e-5-dq3.*dq4.*t6.*8.031412116e-1-dq4.*dq5.*t4.*2.88666e-5-dq3.*dq4.*t8.*1.34574048e-1-dq5.*dq6.*t4.*1.201554327e-3-dq3.*dq5.*t9.*1.1286135e-3-dq4.*dq5.*t9.*1.1286135e-3-dq3.*dq6.*t11.*9.3406347e-3-dq4.*dq6.*t11.*9.3406347e-3+dq3.*dq5.*t56.*2.5575530495e-3+dq4.*dq5.*t56.*2.5575530495e-3-dq3.*dq5.*t148.*2.969136e-6-dq4.*dq5.*t148.*2.969136e-6-dq3.*dq6.*t153.*3.982771635e-4-dq4.*dq6.*t153.*3.982771635e-4+t4.*t8.*t142.*5.07876075e-3+t4.*t8.*t144.*5.07876075e-3-t4.*t10.*t142.*2.1459816e-5-t7.*t8.*t141.*3.1870683e-2-t8.*t9.*t142.*1.298997e-4-t6.*t10.*t144.*4.03054785e-3-t6.*t10.*t145.*4.03054785e-3-t8.*t9.*t144.*1.298997e-4-t9.*t11.*t142.*4.67031735e-3-t9.*t11.*t145.*4.67031735e-3+t6.*t141.*t147.*6.7287024e-2+t6.*t141.*t149.*4.015706058e-1-t8.*t141.*t147.*4.015706058e-1+t8.*t141.*t149.*6.7287024e-2-t9.*t142.*t153.*3.982771635e-4-t141.*t147.*t150.*1.63779518082625e-1-t141.*t147.*t151.*4.520441246e-2+t141.*t149.*t150.*4.520441246e-2-t141.*t149.*t151.*1.63779518082625e-1+dq2.*dq5.*t4.*t7.*1.01575215e-2-dq3.*dq5.*t4.*t6.*2.597994e-4+dq3.*dq4.*t4.*t8.*1.01575215e-2-dq4.*dq5.*t4.*t6.*2.597994e-4-dq2.*dq5.*t5.*t8.*1.05591898525e-2-dq2.*dq5.*t6.*t7.*1.05591898525e-2-dq2.*dq5.*t7.*t9.*2.597994e-4-dq3.*dq4.*t6.*t10.*8.0610957e-3-dq3.*dq5.*t6.*t9.*1.01575215e-2-dq3.*dq4.*t8.*t9.*2.597994e-4-dq4.*dq5.*t6.*t9.*1.01575215e-2-dq5.*dq6.*t4.*t10.*9.3406347e-3+dq3.*dq6.*t8.*t11.*8.0610957e-3-dq3.*dq6.*t9.*t10.*8.956773e-4+dq4.*dq6.*t8.*t11.*8.0610957e-3-dq4.*dq6.*t9.*t10.*8.956773e-4+dq3.*dq6.*t10.*t56.*2.1459816e-5+dq4.*dq6.*t10.*t56.*2.1459816e-5+dq3.*dq5.*t11.*t148.*4.2919632e-5+dq4.*dq5.*t11.*t148.*4.2919632e-5-dq5.*dq6.*t4.*t154.*7.96554327e-4+dq3.*dq5.*t56.*t154.*3.982771635e-4+dq4.*dq5.*t56.*t154.*3.982771635e-4+dq3.*dq6.*t148.*t153.*3.982771635e-4+dq4.*dq6.*t148.*t153.*3.982771635e-4-t4.*t5.*t8.*t141.*4.0307625e-4-t4.*t6.*t7.*t141.*4.0307625e-4-t7.*t8.*t10.*t141.*3.1988475e-4+t8.*t9.*t11.*t142.*4.03054785e-3+t8.*t9.*t11.*t144.*4.03054785e-3+t8.*t9.*t11.*t145.*4.03054785e-3-t4.*t6.*t141.*t147.*5.07876075e-3-t4.*t8.*t141.*t149.*5.07876075e-3+t6.*t9.*t141.*t147.*1.298997e-4+t6.*t10.*t141.*t149.*4.03054785e-3-t8.*t10.*t141.*t147.*4.03054785e-3+t8.*t9.*t141.*t149.*1.298997e-4-t4.*t141.*t147.*t150.*5.6430675e-4+t4.*t141.*t147.*t151.*4.194107562e-3-t4.*t141.*t149.*t150.*4.194107562e-3-t4.*t141.*t149.*t151.*5.6430675e-4+t9.*t141.*t147.*t150.*1.44333e-5-t9.*t141.*t147.*t151.*9.5218542e-5-t10.*t141.*t147.*t150.*4.67031735e-3+t9.*t141.*t149.*t150.*9.5218542e-5-t10.*t141.*t147.*t151.*4.4783865e-4+t9.*t141.*t149.*t151.*1.44333e-5+t10.*t141.*t149.*t150.*4.4783865e-4-t10.*t141.*t149.*t151.*4.67031735e-3-t56.*t141.*t147.*t150.*7.42284e-7-t56.*t141.*t149.*t151.*7.42284e-7-t141.*t147.*t148.*t150.*6.39388262375e-4-t141.*t148.*t149.*t151.*6.39388262375e-4-t141.*t147.*t150.*t154.*2.98707872625e-4-t141.*t149.*t151.*t154.*2.98707872625e-4+dq2.*dq6.*t4.*t5.*t6.*1.201554327e-3-dq2.*dq5.*t4.*t7.*t8.*8.388215124e-3-dq2.*dq5.*t5.*t6.*t9.*1.90437084e-4-dq2.*dq6.*t4.*t7.*t8.*1.201554327e-3-dq2.*dq5.*t5.*t8.*t9.*2.88666e-5-dq2.*dq5.*t6.*t7.*t9.*2.88666e-5+dq2.*dq6.*t4.*t7.*t10.*8.0610957e-3+dq3.*dq5.*t4.*t6.*t11.*8.0610957e-3+dq4.*dq5.*t4.*t6.*t11.*8.0610957e-3-dq2.*dq6.*t5.*t8.*t10.*2.1459816e-5-dq2.*dq6.*t6.*t7.*t10.*2.1459816e-5-dq2.*dq7.*t5.*t8.*t10.*5.0e-6-dq2.*dq7.*t6.*t7.*t10.*5.0e-6+dq5.*dq6.*t4.*t8.*t10.*8.0610957e-3+dq2.*dq5.*t7.*t9.*t11.*8.0610957e-3-dq3.*dq6.*t6.*t9.*t10.*8.0610957e-3+dq3.*dq4.*t8.*t9.*t11.*8.0610957e-3-dq4.*dq6.*t6.*t9.*t10.*8.0610957e-3+dq2.*dq5.*t5.*t8.*t56.*2.969136e-6+dq2.*dq5.*t6.*t7.*t56.*2.969136e-6+dq2.*dq5.*t5.*t8.*t148.*2.5575530495e-3+dq2.*dq5.*t6.*t7.*t148.*2.5575530495e-3+dq2.*dq5.*t5.*t8.*t154.*3.982771635e-4+dq2.*dq5.*t6.*t7.*t154.*3.982771635e-4-t5.*t8.*t9.*t11.*t141.*3.1988475e-4-t6.*t7.*t9.*t11.*t141.*3.1988475e-4-t6.*t9.*t11.*t141.*t147.*4.03054785e-3-t8.*t9.*t11.*t141.*t149.*4.03054785e-3+t4.*t10.*t141.*t147.*t151.*2.1459816e-5-t4.*t10.*t141.*t149.*t150.*2.1459816e-5-t9.*t11.*t141.*t147.*t150.*4.4783865e-4+t9.*t11.*t141.*t147.*t151.*4.67031735e-3-t9.*t11.*t141.*t149.*t150.*4.67031735e-3-t9.*t11.*t141.*t149.*t151.*4.4783865e-4+t11.*t56.*t141.*t147.*t150.*1.0729908e-5+t11.*t56.*t141.*t149.*t151.*1.0729908e-5+t9.*t141.*t147.*t151.*t153.*3.982771635e-4-t9.*t141.*t149.*t150.*t153.*3.982771635e-4-t141.*t147.*t148.*t150.*t154.*9.9569290875e-5-t141.*t148.*t149.*t151.*t154.*9.9569290875e-5-dq2.*dq5.*t4.*t7.*t8.*t10.*4.2919632e-5-dq2.*dq6.*t4.*t7.*t8.*t10.*9.3406347e-3-dq2.*dq7.*t5.*t6.*t9.*t11.*5.0e-6-dq2.*dq5.*t7.*t8.*t9.*t11.*9.3406347e-3-dq2.*dq5.*t5.*t8.*t11.*t56.*4.2919632e-5-dq2.*dq5.*t6.*t7.*t11.*t56.*4.2919632e-5+dq2.*dq6.*t4.*t5.*t6.*t154.*7.96554327e-4+dq2.*dq6.*t5.*t8.*t10.*t148.*2.1459816e-5+dq2.*dq6.*t6.*t7.*t10.*t148.*2.1459816e-5+dq2.*dq5.*t5.*t6.*t9.*t153.*7.96554327e-4-dq2.*dq6.*t4.*t7.*t8.*t154.*7.96554327e-4-dq2.*dq5.*t7.*t8.*t9.*t153.*7.96554327e-4-dq2.*dq6.*t5.*t8.*t56.*t153.*3.982771635e-4-dq2.*dq6.*t6.*t7.*t56.*t153.*3.982771635e-4+dq2.*dq5.*t5.*t8.*t148.*t154.*3.982771635e-4+dq2.*dq5.*t6.*t7.*t148.*t154.*3.982771635e-4,t141.*4.520441246e-2+t155+t156+t157+t158+t159+t160+t161+t162+t163+t164+t165+t166+t167+t168+t169+t170+t171+t172+t173+t174+t175+t176+t177+t178+dq3.*dq5.*2.969136e-6+dq4.*dq5.*2.969136e-6-t4.*t141.*4.194107562e-3-t4.*t142.*4.194107562e-3+t6.*t143.*4.015706058e-1+t9.*t141.*9.5218542e-5+t8.*t143.*6.7287024e-2+t10.*t141.*4.4783865e-4-t10.*t145.*4.4783865e-4-t23.*t141.*9.040882492e-2-t24.*t141.*9.040882492e-2+t141.*t147.*1.629409912385e-1+t141.*t151.*1.629409912385e-1-dq3.*dq5.*t4.*2.88666e-5-dq4.*dq5.*t4.*2.88666e-5-dq5.*dq6.*t4.*4.05e-4-dq3.*dq5.*t9.*1.1286135e-3-dq4.*dq5.*t9.*1.1286135e-3-dq3.*dq5.*t11.*4.2919632e-5-dq3.*dq6.*t11.*9.3406347e-3-dq4.*dq5.*t11.*4.2919632e-5-dq4.*dq6.*t11.*9.3406347e-3-dq3.*dq5.*t26.*5.938272e-6-dq4.*dq5.*t26.*5.938272e-6+dq3.*dq5.*t56.*2.159275886e-3+dq4.*dq5.*t56.*2.159275886e-3-dq3.*dq6.*t153.*7.96554327e-4-dq4.*dq6.*t153.*7.96554327e-4-t4.*t8.*t143.*5.07876075e-3-t4.*t10.*t141.*2.1459816e-5-t4.*t10.*t142.*2.1459816e-5-t7.*t8.*t141.*3.1870683e-2+t6.*t10.*t143.*4.03054785e-3+t8.*t9.*t143.*1.298997e-4-t9.*t11.*t141.*4.67031735e-3-t9.*t11.*t142.*4.67031735e-3-t9.*t11.*t145.*4.67031735e-3+t4.*t23.*t141.*8.388215124e-3+t4.*t24.*t141.*8.388215124e-3+t6.*t23.*t141.*4.015706058e-1+t8.*t23.*t141.*6.7287024e-2-t9.*t23.*t141.*1.90437084e-4-t9.*t24.*t141.*1.90437084e-4-t10.*t23.*t141.*8.956773e-4-t10.*t24.*t141.*8.956773e-4+t23.*t24.*t141.*1.8081764984e-1-dq2.*dq5.*t5.*t8.*1.3116742902e-2-dq2.*dq5.*t6.*t7.*1.3116742902e-2-dq5.*dq6.*t4.*t10.*9.3406347e-3-dq3.*dq6.*t9.*t10.*8.956773e-4-dq4.*dq6.*t9.*t10.*8.956773e-4-dq5.*dq6.*t4.*t25.*1.593108654e-3+dq3.*dq5.*t11.*t26.*8.5839264e-5+dq4.*dq5.*t11.*t26.*8.5839264e-5+t4.*t5.*t7.*t141.*1.1286135e-3-t4.*t5.*t8.*t141.*4.0307625e-4-t4.*t6.*t7.*t141.*4.0307625e-4+t4.*t6.*t8.*t141.*1.1286135e-3+t5.*t6.*t7.*t141.*6.7287024e-2-t5.*t7.*t8.*t141.*4.015706058e-1-t5.*t7.*t9.*t141.*2.88666e-5+t5.*t7.*t10.*t141.*9.3406347e-3-t6.*t8.*t9.*t141.*2.88666e-5+t6.*t8.*t10.*t141.*9.3406347e-3-t7.*t8.*t10.*t141.*3.1988475e-4-t8.*t9.*t11.*t143.*4.03054785e-3-t9.*t10.*t11.*t141.*7.96554327e-4-t9.*t10.*t11.*t142.*7.96554327e-4-t4.*t8.*t23.*t141.*5.07876075e-3-t5.*t7.*t24.*t141.*6.51763964954e-1+t4.*t10.*t23.*t141.*4.2919632e-5+t5.*t7.*t25.*t141.*7.96554327e-4-t6.*t8.*t23.*t141.*6.51763964954e-1+t4.*t10.*t24.*t141.*4.2919632e-5+t5.*t7.*t26.*t141.*2.159275886e-3+t6.*t8.*t25.*t141.*7.96554327e-4+t6.*t10.*t23.*t141.*4.03054785e-3+t6.*t8.*t26.*t141.*2.159275886e-3+t8.*t9.*t23.*t141.*1.298997e-4+t9.*t11.*t23.*t141.*9.3406347e-3+t9.*t11.*t24.*t141.*9.3406347e-3-t4.*t23.*t24.*t141.*1.6776430248e-2+t9.*t23.*t24.*t141.*3.80874168e-4+t10.*t23.*t24.*t141.*1.7913546e-3+dq2.*dq6.*t4.*t5.*t6.*4.05e-4-dq2.*dq5.*t4.*t7.*t8.*8.388215124e-3-dq2.*dq5.*t5.*t6.*t9.*1.90437084e-4-dq2.*dq6.*t4.*t7.*t8.*4.05e-4-dq2.*dq5.*t5.*t8.*t9.*2.88666e-5-dq2.*dq5.*t6.*t7.*t9.*2.88666e-5-dq2.*dq6.*t5.*t8.*t10.*4.2919632e-5-dq2.*dq6.*t6.*t7.*t10.*4.2919632e-5-dq2.*dq7.*t5.*t8.*t10.*5.0e-6-dq2.*dq7.*t6.*t7.*t10.*5.0e-6+dq3.*dq6.*t4.*t9.*t10.*4.2919632e-5+dq4.*dq6.*t4.*t9.*t10.*4.2919632e-5+dq2.*dq5.*t5.*t8.*t26.*4.318551772e-3+dq2.*dq5.*t6.*t7.*t26.*4.318551772e-3+dq3.*dq5.*t4.*t9.*t25.*1.593108654e-3+dq4.*dq5.*t4.*t9.*t25.*1.593108654e-3+dq3.*dq6.*t10.*t11.*t26.*1.593108654e-3+dq4.*dq6.*t10.*t11.*t26.*1.593108654e-3-t4.*t5.*t6.*t7.*t141.*5.07876075e-3+t4.*t5.*t7.*t9.*t141.*2.969136e-6-t5.*t6.*t7.*t8.*t141.*1.8081764984e-1+t4.*t6.*t8.*t9.*t141.*2.969136e-6+t5.*t6.*t7.*t9.*t141.*1.298997e-4-t5.*t7.*t8.*t10.*t141.*4.03054785e-3+t5.*t7.*t9.*t11.*t141.*8.956773e-4-t5.*t8.*t9.*t11.*t141.*3.1988475e-4-t6.*t7.*t9.*t11.*t141.*3.1988475e-4+t6.*t8.*t9.*t11.*t141.*8.956773e-4-t4.*t5.*t7.*t24.*t141.*2.257227e-3-t4.*t6.*t8.*t23.*t141.*2.257227e-3+t5.*t7.*t9.*t24.*t141.*5.77332e-5-t5.*t7.*t10.*t24.*t141.*1.86812694e-2+t6.*t8.*t9.*t23.*t141.*5.77332e-5-t6.*t8.*t10.*t23.*t141.*1.86812694e-2-t8.*t9.*t11.*t23.*t141.*4.03054785e-3+t9.*t10.*t11.*t23.*t141.*1.593108654e-3+t9.*t10.*t11.*t24.*t141.*1.593108654e-3-t4.*t10.*t23.*t24.*t141.*8.5839264e-5-t5.*t7.*t24.*t25.*t141.*1.593108654e-3-t5.*t7.*t24.*t26.*t141.*4.318551772e-3-t6.*t8.*t23.*t25.*t141.*1.593108654e-3+t5.*t7.*t25.*t26.*t141.*7.96554327e-4-t6.*t8.*t23.*t26.*t141.*4.318551772e-3+t6.*t8.*t25.*t26.*t141.*7.96554327e-4-t9.*t11.*t23.*t24.*t141.*1.86812694e-2+t4.*t5.*t6.*t7.*t8.*t141.*1.6776430248e-2-t5.*t6.*t7.*t8.*t9.*t141.*3.80874168e-4-t4.*t5.*t7.*t9.*t11.*t141.*4.2919632e-5-t5.*t6.*t7.*t8.*t10.*t141.*1.7913546e-3-t4.*t6.*t8.*t9.*t11.*t141.*4.2919632e-5-t5.*t6.*t7.*t9.*t11.*t141.*4.03054785e-3-t4.*t5.*t7.*t9.*t24.*t141.*5.938272e-6-t4.*t6.*t8.*t9.*t23.*t141.*5.938272e-6-t5.*t7.*t9.*t11.*t24.*t141.*1.7913546e-3-t6.*t8.*t9.*t11.*t23.*t141.*1.7913546e-3-t9.*t10.*t11.*t23.*t24.*t141.*3.186217308e-3-t5.*t7.*t24.*t25.*t26.*t141.*1.593108654e-3-t6.*t8.*t23.*t25.*t26.*t141.*1.593108654e-3+dq2.*dq5.*t4.*t5.*t8.*t9.*5.938272e-6+dq2.*dq5.*t4.*t6.*t7.*t9.*5.938272e-6-dq2.*dq5.*t4.*t7.*t8.*t10.*4.2919632e-5-dq2.*dq6.*t4.*t7.*t8.*t10.*9.3406347e-3-dq2.*dq7.*t5.*t6.*t9.*t11.*5.0e-6-dq2.*dq5.*t7.*t8.*t9.*t11.*9.3406347e-3+dq2.*dq6.*t4.*t5.*t6.*t25.*1.593108654e-3-dq2.*dq6.*t4.*t7.*t8.*t25.*1.593108654e-3+dq2.*dq6.*t5.*t8.*t10.*t26.*4.2919632e-5+dq2.*dq6.*t6.*t7.*t10.*t26.*4.2919632e-5+dq2.*dq5.*t5.*t8.*t25.*t26.*1.593108654e-3+dq2.*dq5.*t6.*t7.*t25.*t26.*1.593108654e-3-dq2.*dq5.*t4.*t5.*t8.*t9.*t11.*8.5839264e-5-dq2.*dq5.*t4.*t6.*t7.*t9.*t11.*8.5839264e-5+dq2.*dq5.*t5.*t6.*t9.*t10.*t11.*1.593108654e-3-dq2.*dq5.*t7.*t8.*t9.*t10.*t11.*1.593108654e-3+t4.*t5.*t6.*t7.*t8.*t10.*t141.*8.5839264e-5+t5.*t6.*t7.*t8.*t9.*t11.*t141.*1.86812694e-2+t4.*t5.*t7.*t9.*t11.*t24.*t141.*8.5839264e-5+t4.*t6.*t8.*t9.*t11.*t23.*t141.*8.5839264e-5-dq2.*dq6.*t4.*t5.*t8.*t9.*t10.*t11.*1.593108654e-3-dq2.*dq6.*t4.*t6.*t7.*t9.*t10.*t11.*1.593108654e-3+t5.*t6.*t7.*t8.*t9.*t10.*t11.*t141.*3.186217308e-3,t143.*(-1.484568e-6)-t144.*1.484568e-6-dq3.*dq4.*2.969136e-6+t4.*t141.*1.44333e-5+t4.*t143.*1.44333e-5+t4.*t144.*1.44333e-5+t9.*t141.*5.6430675e-4+t9.*t143.*5.6430675e-4+t9.*t144.*5.6430675e-4+t11.*t143.*2.1459816e-5+t11.*t144.*2.1459816e-5-t11.*t145.*2.1459816e-5+t23.*t141.*1.484568e-6+t24.*t141.*1.484568e-6+t26.*t143.*2.969136e-6+t26.*t144.*2.969136e-6-t56.*t143.*1.079637943e-3-t56.*t144.*1.079637943e-3+dq3.*dq4.*t4.*2.88666e-5+dq3.*dq6.*t4.*1.998108654e-3+dq4.*dq6.*t4.*1.998108654e-3+dq3.*dq4.*t9.*1.1286135e-3+dq3.*dq4.*t11.*4.2919632e-5-dq6.*dq7.*t11.*5.0e-6+dq3.*dq4.*t26.*5.938272e-6-dq3.*dq4.*t56.*2.159275886e-3+dq5.*dq6.*t153.*7.96554327e-4+t4.*t6.*t143.*1.298997e-4-t4.*t11.*t141.*4.4783865e-4-t4.*t11.*t143.*4.4783865e-4+t6.*t9.*t143.*5.07876075e-3-t4.*t11.*t144.*4.4783865e-4-t4.*t23.*t141.*1.44333e-5-t4.*t24.*t141.*1.44333e-5-t9.*t23.*t141.*5.6430675e-4-t9.*t24.*t141.*5.6430675e-4-t11.*t23.*t141.*2.1459816e-5-t11.*t24.*t141.*2.1459816e-5-t11.*t26.*t143.*4.2919632e-5-t11.*t26.*t144.*4.2919632e-5-t23.*t24.*t141.*2.969136e-6-t23.*t26.*t141.*2.969136e-6-t24.*t26.*t141.*2.969136e-6-dq2.*dq3.*t4.*t7.*1.01575215e-2+dq2.*dq3.*t5.*t8.*1.3116742902e-2+dq2.*dq3.*t6.*t7.*1.3116742902e-2+dq2.*dq4.*t5.*t8.*1.3116742902e-2+dq2.*dq4.*t6.*t7.*1.3116742902e-2+dq2.*dq3.*t7.*t9.*2.597994e-4-dq3.*dq4.*t4.*t11.*8.956773e-4-dq3.*dq6.*t9.*t11.*4.2919632e-5-dq3.*dq7.*t9.*t11.*5.0e-6-dq4.*dq6.*t9.*t11.*4.2919632e-5-dq4.*dq7.*t9.*t11.*5.0e-6-dq3.*dq6.*t4.*t25.*1.593108654e-3-dq4.*dq6.*t4.*t25.*1.593108654e-3-dq3.*dq4.*t11.*t26.*8.5839264e-5+t4.*t5.*t6.*t141.*1.03095e-5+t4.*t5.*t7.*t141.*9.5218542e-5+t4.*t6.*t8.*t141.*9.5218542e-5-t4.*t7.*t8.*t141.*1.03095e-5+t5.*t6.*t9.*t141.*4.0307625e-4+t5.*t7.*t9.*t141.*4.194107562e-3-t4.*t6.*t11.*t143.*4.03054785e-3+t6.*t8.*t9.*t141.*4.194107562e-3-t7.*t8.*t9.*t141.*4.0307625e-4+t4.*t6.*t23.*t141.*1.298997e-4+t4.*t9.*t23.*t141.*2.159275886e-3+t4.*t9.*t24.*t141.*2.159275886e-3+t4.*t11.*t23.*t141.*4.4783865e-4+t6.*t9.*t23.*t141.*5.07876075e-3+t4.*t11.*t24.*t141.*4.4783865e-4-t4.*t9.*t25.*t143.*7.96554327e-4-t4.*t9.*t25.*t144.*7.96554327e-4+t4.*t23.*t24.*t141.*2.88666e-5+t9.*t23.*t24.*t141.*1.1286135e-3+t11.*t23.*t24.*t141.*4.2919632e-5+t11.*t23.*t26.*t141.*4.2919632e-5+t11.*t24.*t26.*t141.*4.2919632e-5+t23.*t24.*t26.*t141.*5.938272e-6-dq2.*dq3.*t4.*t5.*t6.*8.388215124e-3-dq2.*dq4.*t4.*t5.*t6.*8.388215124e-3-dq2.*dq3.*t4.*t5.*t8.*1.1286135e-3-dq2.*dq3.*t4.*t6.*t7.*1.1286135e-3-dq2.*dq4.*t4.*t5.*t8.*1.1286135e-3-dq2.*dq4.*t4.*t6.*t7.*1.1286135e-3+dq2.*dq3.*t4.*t7.*t8.*8.388215124e-3+dq2.*dq3.*t5.*t6.*t9.*1.90437084e-4+dq2.*dq4.*t4.*t7.*t8.*8.388215124e-3+dq2.*dq4.*t5.*t6.*t9.*1.90437084e-4+dq2.*dq3.*t5.*t8.*t9.*2.88666e-5+dq2.*dq3.*t6.*t7.*t9.*2.88666e-5+dq2.*dq4.*t5.*t8.*t9.*2.88666e-5+dq2.*dq4.*t6.*t7.*t9.*2.88666e-5-dq2.*dq3.*t7.*t8.*t9.*1.90437084e-4-dq2.*dq4.*t7.*t8.*t9.*1.90437084e-4+dq2.*dq6.*t5.*t8.*t9.*1.998108654e-3+dq2.*dq6.*t6.*t7.*t9.*1.998108654e-3-dq2.*dq3.*t7.*t9.*t11.*8.0610957e-3-dq2.*dq3.*t5.*t8.*t26.*4.318551772e-3-dq2.*dq3.*t6.*t7.*t26.*4.318551772e-3-dq2.*dq4.*t5.*t8.*t26.*4.318551772e-3-dq2.*dq4.*t6.*t7.*t26.*4.318551772e-3-dq3.*dq4.*t4.*t9.*t25.*1.593108654e-3-t4.*t5.*t7.*t8.*t141.*1.298997e-4-t4.*t5.*t6.*t11.*t141.*3.1988475e-4+t5.*t6.*t7.*t8.*t141.*2.969136e-6-t4.*t5.*t7.*t11.*t141.*4.67031735e-3-t4.*t6.*t8.*t11.*t141.*4.67031735e-3-t5.*t7.*t8.*t9.*t141.*5.07876075e-3+t4.*t7.*t8.*t11.*t141.*3.1988475e-4+t5.*t7.*t9.*t10.*t141.*2.1459816e-5+t6.*t8.*t9.*t10.*t141.*2.1459816e-5-t4.*t5.*t7.*t24.*t141.*1.90437084e-4-t4.*t6.*t8.*t23.*t141.*1.90437084e-4-t4.*t6.*t11.*t23.*t141.*4.03054785e-3-t5.*t7.*t9.*t24.*t141.*8.388215124e-3-t6.*t8.*t9.*t23.*t141.*8.388215124e-3-t4.*t9.*t23.*t24.*t141.*4.318551772e-3+t4.*t9.*t23.*t25.*t141.*7.96554327e-4+t4.*t9.*t24.*t25.*t141.*7.96554327e-4-t4.*t11.*t23.*t24.*t141.*8.956773e-4-t11.*t23.*t24.*t26.*t141.*8.5839264e-5-t4.*t5.*t6.*t7.*t8.*t141.*2.88666e-5+t4.*t5.*t7.*t8.*t11.*t141.*4.03054785e-3-t5.*t6.*t7.*t8.*t9.*t141.*1.1286135e-3-t4.*t5.*t7.*t10.*t11.*t141.*7.96554327e-4-t5.*t6.*t7.*t8.*t11.*t141.*4.2919632e-5-t4.*t6.*t8.*t10.*t11.*t141.*7.96554327e-4+t4.*t5.*t7.*t11.*t24.*t141.*9.3406347e-3+t4.*t6.*t8.*t11.*t23.*t141.*9.3406347e-3-t5.*t6.*t7.*t8.*t26.*t141.*5.938272e-6-t5.*t7.*t9.*t10.*t24.*t141.*4.2919632e-5-t6.*t8.*t9.*t10.*t23.*t141.*4.2919632e-5-t4.*t9.*t23.*t24.*t25.*t141.*1.593108654e-3-dq2.*dq3.*t4.*t5.*t6.*t10.*4.2919632e-5-dq2.*dq3.*t4.*t5.*t8.*t9.*5.938272e-6-dq2.*dq3.*t4.*t6.*t7.*t9.*5.938272e-6-dq2.*dq4.*t4.*t5.*t6.*t10.*4.2919632e-5-dq2.*dq4.*t4.*t5.*t8.*t9.*5.938272e-6-dq2.*dq4.*t4.*t6.*t7.*t9.*5.938272e-6+dq2.*dq3.*t4.*t7.*t8.*t10.*4.2919632e-5+dq2.*dq4.*t4.*t7.*t8.*t10.*4.2919632e-5-dq2.*dq3.*t5.*t6.*t9.*t11.*9.3406347e-3+dq2.*dq6.*t4.*t5.*t8.*t11.*4.2919632e-5+dq2.*dq6.*t4.*t6.*t7.*t11.*4.2919632e-5-dq2.*dq4.*t5.*t6.*t9.*t11.*9.3406347e-3+dq2.*dq7.*t4.*t5.*t8.*t11.*5.0e-6+dq2.*dq7.*t4.*t6.*t7.*t11.*5.0e-6-dq2.*dq3.*t5.*t8.*t9.*t11.*8.956773e-4-dq2.*dq3.*t6.*t7.*t9.*t11.*8.956773e-4-dq2.*dq4.*t5.*t8.*t9.*t11.*8.956773e-4-dq2.*dq4.*t6.*t7.*t9.*t11.*8.956773e-4+dq2.*dq3.*t7.*t8.*t9.*t11.*9.3406347e-3-dq2.*dq6.*t5.*t6.*t10.*t11.*1.593108654e-3+dq2.*dq4.*t7.*t8.*t9.*t11.*9.3406347e-3+dq2.*dq6.*t7.*t8.*t10.*t11.*1.593108654e-3-dq2.*dq6.*t5.*t8.*t9.*t25.*1.593108654e-3-dq2.*dq6.*t6.*t7.*t9.*t25.*1.593108654e-3-dq2.*dq3.*t5.*t8.*t25.*t26.*1.593108654e-3-dq2.*dq3.*t6.*t7.*t25.*t26.*1.593108654e-3-dq2.*dq4.*t5.*t8.*t25.*t26.*1.593108654e-3-dq2.*dq4.*t6.*t7.*t25.*t26.*1.593108654e-3+dq2.*dq3.*t4.*t5.*t8.*t9.*t11.*8.5839264e-5+dq2.*dq3.*t4.*t6.*t7.*t9.*t11.*8.5839264e-5+dq2.*dq4.*t4.*t5.*t8.*t9.*t11.*8.5839264e-5+dq2.*dq4.*t4.*t6.*t7.*t9.*t11.*8.5839264e-5-dq2.*dq3.*t5.*t6.*t9.*t10.*t11.*1.593108654e-3-dq2.*dq4.*t5.*t6.*t9.*t10.*t11.*1.593108654e-3+dq2.*dq3.*t7.*t8.*t9.*t10.*t11.*1.593108654e-3+dq2.*dq4.*t7.*t8.*t9.*t10.*t11.*1.593108654e-3+t4.*t5.*t6.*t7.*t8.*t9.*t141.*4.318551772e-3+t4.*t5.*t6.*t7.*t8.*t11.*t141.*8.956773e-4+t4.*t5.*t7.*t10.*t11.*t24.*t141.*1.593108654e-3+t4.*t6.*t8.*t10.*t11.*t23.*t141.*1.593108654e-3+t5.*t6.*t7.*t8.*t11.*t26.*t141.*8.5839264e-5+t4.*t5.*t6.*t7.*t8.*t9.*t25.*t141.*1.593108654e-3,t11.*t143.*4.67031735e-3+t11.*t144.*4.67031735e-3-t141.*t153.*3.982771635e-4-t142.*t153.*3.982771635e-4+t143.*t153.*3.982771635e-4+t144.*t153.*3.982771635e-4-dq3.*dq5.*t4.*1.998108654e-3-dq4.*dq5.*t4.*1.998108654e-3+dq3.*dq4.*t11.*9.3406347e-3+dq5.*dq7.*t11.*5.0e-6+dq3.*dq4.*t153.*7.96554327e-4+t9.*t10.*t141.*4.4783865e-4-t8.*t11.*t143.*4.03054785e-3+t9.*t10.*t143.*4.4783865e-4+t9.*t10.*t144.*4.4783865e-4+t11.*t23.*t141.*4.67031735e-3+t11.*t24.*t141.*4.67031735e-3-dq3.*dq7.*t4.*t10.*5.0e-6-dq4.*dq7.*t4.*t10.*5.0e-6+dq3.*dq4.*t9.*t10.*8.956773e-4+dq3.*dq5.*t9.*t11.*4.2919632e-5+dq4.*dq5.*t9.*t11.*4.2919632e-5+dq3.*dq5.*t4.*t25.*1.593108654e-3+dq4.*dq5.*t4.*t25.*1.593108654e-3-t5.*t7.*t9.*t141.*7.96554327e-4+t5.*t7.*t11.*t141.*4.4783865e-4-t6.*t8.*t9.*t141.*7.96554327e-4-t5.*t8.*t11.*t141.*3.1988475e-4-t6.*t7.*t11.*t141.*3.1988475e-4-t4.*t9.*t10.*t143.*2.1459816e-5+t6.*t8.*t11.*t141.*4.4783865e-4-t4.*t9.*t10.*t144.*2.1459816e-5+t6.*t9.*t10.*t143.*4.03054785e-3-t8.*t11.*t23.*t141.*4.03054785e-3-t9.*t10.*t23.*t141.*4.4783865e-4-t9.*t10.*t24.*t141.*4.4783865e-4+t10.*t11.*t23.*t141.*7.96554327e-4+t10.*t11.*t24.*t141.*7.96554327e-4-t10.*t11.*t26.*t143.*7.96554327e-4-t10.*t11.*t26.*t144.*7.96554327e-4-t11.*t23.*t24.*t141.*9.3406347e-3-dq2.*dq3.*t4.*t5.*t6.*4.05e-4-dq2.*dq4.*t4.*t5.*t6.*4.05e-4+dq2.*dq3.*t4.*t7.*t8.*4.05e-4+dq2.*dq4.*t4.*t7.*t8.*4.05e-4-dq2.*dq3.*t4.*t7.*t10.*8.0610957e-3+dq2.*dq3.*t5.*t8.*t10.*4.2919632e-5+dq2.*dq3.*t6.*t7.*t10.*4.2919632e-5+dq2.*dq4.*t5.*t8.*t10.*4.2919632e-5+dq2.*dq4.*t6.*t7.*t10.*4.2919632e-5-dq2.*dq5.*t5.*t8.*t9.*1.998108654e-3-dq2.*dq5.*t6.*t7.*t9.*1.998108654e-3-dq3.*dq4.*t4.*t9.*t10.*4.2919632e-5-dq2.*dq7.*t5.*t6.*t11.*5.0e-6+dq2.*dq7.*t7.*t8.*t11.*5.0e-6-dq3.*dq4.*t10.*t11.*t26.*1.593108654e-3-t4.*t5.*t7.*t11.*t141.*2.1459816e-5-t4.*t6.*t8.*t11.*t141.*2.1459816e-5-t5.*t6.*t7.*t11.*t141.*4.03054785e-3+t5.*t6.*t9.*t10.*t141.*3.1988475e-4+t5.*t7.*t9.*t10.*t141.*4.67031735e-3+t6.*t8.*t9.*t10.*t141.*4.67031735e-3-t7.*t8.*t9.*t10.*t141.*3.1988475e-4+t5.*t7.*t9.*t24.*t141.*1.593108654e-3+t4.*t9.*t10.*t23.*t141.*2.1459816e-5+t5.*t7.*t9.*t25.*t141.*1.593108654e-3+t6.*t8.*t9.*t23.*t141.*1.593108654e-3+t4.*t9.*t10.*t24.*t141.*2.1459816e-5-t5.*t7.*t11.*t24.*t141.*8.956773e-4+t6.*t8.*t9.*t25.*t141.*1.593108654e-3-t6.*t8.*t11.*t23.*t141.*8.956773e-4+t6.*t9.*t10.*t23.*t141.*4.03054785e-3+t9.*t10.*t23.*t24.*t141.*8.956773e-4-t10.*t11.*t23.*t24.*t141.*1.593108654e-3+t10.*t11.*t23.*t26.*t141.*7.96554327e-4+t10.*t11.*t24.*t26.*t141.*7.96554327e-4+t5.*t6.*t7.*t8.*t11.*t141.*9.3406347e-3-t5.*t7.*t8.*t9.*t10.*t141.*4.03054785e-3+t4.*t5.*t7.*t11.*t24.*t141.*4.2919632e-5+t4.*t6.*t8.*t11.*t23.*t141.*4.2919632e-5-t5.*t7.*t9.*t10.*t24.*t141.*9.3406347e-3-t6.*t8.*t9.*t10.*t23.*t141.*9.3406347e-3-t4.*t9.*t10.*t23.*t24.*t141.*4.2919632e-5-t5.*t7.*t9.*t24.*t25.*t141.*3.186217308e-3-t6.*t8.*t9.*t23.*t25.*t141.*3.186217308e-3-t10.*t11.*t23.*t24.*t26.*t141.*1.593108654e-3-dq2.*dq3.*t4.*t5.*t6.*t10.*9.3406347e-3-dq2.*dq4.*t4.*t5.*t6.*t10.*9.3406347e-3-dq2.*dq3.*t4.*t5.*t8.*t10.*8.956773e-4-dq2.*dq3.*t4.*t6.*t7.*t10.*8.956773e-4-dq2.*dq4.*t4.*t5.*t8.*t10.*8.956773e-4-dq2.*dq4.*t4.*t6.*t7.*t10.*8.956773e-4+dq2.*dq3.*t4.*t7.*t8.*t10.*9.3406347e-3+dq2.*dq4.*t4.*t7.*t8.*t10.*9.3406347e-3-dq2.*dq5.*t4.*t5.*t8.*t11.*4.2919632e-5-dq2.*dq5.*t4.*t6.*t7.*t11.*4.2919632e-5+dq2.*dq5.*t5.*t6.*t10.*t11.*1.593108654e-3-dq2.*dq7.*t5.*t8.*t9.*t10.*5.0e-6-dq2.*dq7.*t6.*t7.*t9.*t10.*5.0e-6-dq2.*dq5.*t7.*t8.*t10.*t11.*1.593108654e-3-dq2.*dq3.*t4.*t5.*t6.*t25.*1.593108654e-3-dq2.*dq4.*t4.*t5.*t6.*t25.*1.593108654e-3+dq2.*dq3.*t4.*t7.*t8.*t25.*1.593108654e-3+dq2.*dq4.*t4.*t7.*t8.*t25.*1.593108654e-3-dq2.*dq3.*t5.*t8.*t10.*t26.*4.2919632e-5-dq2.*dq3.*t6.*t7.*t10.*t26.*4.2919632e-5+dq2.*dq5.*t5.*t8.*t9.*t25.*1.593108654e-3+dq2.*dq5.*t6.*t7.*t9.*t25.*1.593108654e-3-dq2.*dq4.*t5.*t8.*t10.*t26.*4.2919632e-5-dq2.*dq4.*t6.*t7.*t10.*t26.*4.2919632e-5-t5.*t6.*t7.*t8.*t9.*t10.*t141.*8.956773e-4+t5.*t6.*t7.*t8.*t10.*t11.*t141.*1.593108654e-3+dq2.*dq3.*t4.*t5.*t8.*t9.*t10.*t11.*1.593108654e-3+dq2.*dq3.*t4.*t6.*t7.*t9.*t10.*t11.*1.593108654e-3+dq2.*dq4.*t4.*t5.*t8.*t9.*t10.*t11.*1.593108654e-3+dq2.*dq4.*t4.*t6.*t7.*t9.*t10.*t11.*1.593108654e-3+t4.*t5.*t6.*t7.*t8.*t9.*t10.*t141.*4.2919632e-5+t5.*t6.*t7.*t8.*t10.*t11.*t26.*t141.*1.593108654e-3,dq5.*dq6.*t11.*(-5.0e-6)+dq3.*dq6.*t4.*t10.*5.0e-6+dq4.*dq6.*t4.*t10.*5.0e-6+dq3.*dq5.*t9.*t11.*5.0e-6+dq4.*dq5.*t9.*t11.*5.0e-6+dq2.*dq3.*t5.*t8.*t10.*5.0e-6+dq2.*dq3.*t6.*t7.*t10.*5.0e-6+dq2.*dq4.*t5.*t8.*t10.*5.0e-6+dq2.*dq4.*t6.*t7.*t10.*5.0e-6+dq2.*dq6.*t5.*t6.*t11.*5.0e-6-dq2.*dq6.*t7.*t8.*t11.*5.0e-6-dq2.*dq5.*t4.*t5.*t8.*t11.*5.0e-6-dq2.*dq5.*t4.*t6.*t7.*t11.*5.0e-6+dq2.*dq3.*t5.*t6.*t9.*t11.*5.0e-6+dq2.*dq4.*t5.*t6.*t9.*t11.*5.0e-6-dq2.*dq3.*t7.*t8.*t9.*t11.*5.0e-6+dq2.*dq6.*t5.*t8.*t9.*t10.*5.0e-6+dq2.*dq6.*t6.*t7.*t9.*t10.*5.0e-6-dq2.*dq4.*t7.*t8.*t9.*t11.*5.0e-6];
end
if nargout > 3
    t179 = dq2.*dq5.*t7.*(2.1e1./1.0e3);
    t180 = dq6.*dq7.*t4.*t25.*(2.1e1./1.0e3);
    t181 = dq2.*dq7.*t5.*t8.*(2.1e1./1.0e3);
    t182 = dq2.*dq7.*t6.*t7.*(2.1e1./1.0e3);
    t183 = dq5.*dq7.*t4.*t10.*(2.1e1./1.0e3);
    t184 = dq2.*dq6.*t5.*t8.*t9.*(2.1e1./1.0e3);
    t185 = dq2.*dq6.*t6.*t7.*t9.*(2.1e1./1.0e3);
    t186 = dq5.*dq7.*t9.*t10.*t11.*(2.1e1./1.0e3);
    t187 = dq2.*dq6.*t4.*t5.*t6.*t9.*(2.1e1./1.0e3);
    t188 = dq2.*dq7.*t4.*t7.*t8.*t10.*(2.1e1./1.0e3);
    t189 = dq2.*dq7.*t7.*t8.*t9.*t10.*t11.*(2.1e1./1.0e3);
    t190 = t179+t180+t181+t182+t183+t184+t185+t186+t187+t188+t189-dq6.*dq7.*t4.*(2.1e1./1.0e3)-dq5.*dq6.*t56.*1.05e-2-dq2.*dq5.*t7.*t24.*(2.1e1./1.0e3)-dq2.*dq5.*t5.*t6.*t8.*(2.1e1./1.0e3)-dq2.*dq7.*t5.*t8.*t25.*(2.1e1./1.0e3)-dq2.*dq7.*t6.*t7.*t25.*(2.1e1./1.0e3)-dq2.*dq7.*t4.*t5.*t6.*t10.*(2.1e1./1.0e3)-dq2.*dq6.*t4.*t7.*t8.*t9.*(2.1e1./1.0e3)-dq2.*dq7.*t5.*t6.*t9.*t10.*t11.*(2.1e1./1.0e3);
    t191 = dq3+dq4;
    t192 = t4.*t191;
    t193 = dq2.*t9.*t138;
    t194 = t192+t193;
    t197 = dq2.*t139;
    t195 = dq5-t197;
    t196 = t9.*t191;
    t198 = dq3.*t9;
    t199 = dq4.*t9;
    t200 = t198+t199-dq2.*t4.*t138;
    t201 = t10.*t195;
    t202 = dq5+t197;
    t203 = dq3.*(2.1e1./1.0e3);
    t204 = dq4.*(2.1e1./1.0e3);
    t205 = t203+t204;
    t206 = dq3.*t4;
    t207 = dq4.*t4;
    t208 = t193+t206+t207;
    t209 = t11.*t208;
    t210 = t201+t209;
    t211 = dq2.*dq5.*t4.*t138.*(2.1e1./1.0e3);
    t212 = dq2.*t5.*t8.*t191.*(2.1e1./1.0e3);
    t213 = dq2.*t6.*t7.*t191.*(2.1e1./1.0e3);
    phim = [0.0,dq3.*dq5.*t7.*(-2.1e1./1.0e3)-dq4.*dq5.*t7.*(2.1e1./1.0e3)-dq3.*dq7.*t5.*t8.*(2.1e1./1.0e3)-dq3.*dq7.*t6.*t7.*(2.1e1./1.0e3)-dq4.*dq7.*t5.*t8.*(2.1e1./1.0e3)-dq4.*dq7.*t6.*t7.*(2.1e1./1.0e3)+dq5.*dq6.*t5.*t8.*(2.1e1./1.0e3)+dq5.*dq6.*t6.*t7.*(2.1e1./1.0e3)+dq3.*dq5.*t7.*t24.*(2.1e1./1.0e3)+dq4.*dq5.*t7.*t24.*(2.1e1./1.0e3)+dq3.*dq5.*t5.*t6.*t8.*(2.1e1./1.0e3)+dq4.*dq5.*t5.*t6.*t8.*(2.1e1./1.0e3)-dq3.*dq6.*t5.*t8.*t9.*(2.1e1./1.0e3)-dq3.*dq6.*t6.*t7.*t9.*(2.1e1./1.0e3)-dq4.*dq6.*t5.*t8.*t9.*(2.1e1./1.0e3)-dq4.*dq6.*t6.*t7.*t9.*(2.1e1./1.0e3)-dq6.*dq7.*t5.*t8.*t9.*(2.1e1./1.0e3)-dq6.*dq7.*t6.*t7.*t9.*(2.1e1./1.0e3)+dq3.*dq7.*t5.*t8.*t25.*(2.1e1./1.0e3)+dq3.*dq7.*t6.*t7.*t25.*(2.1e1./1.0e3)+dq4.*dq7.*t5.*t8.*t25.*(2.1e1./1.0e3)+dq4.*dq7.*t6.*t7.*t25.*(2.1e1./1.0e3)-dq5.*dq6.*t5.*t8.*t26.*(2.1e1./1.0e3)-dq5.*dq6.*t6.*t7.*t26.*(2.1e1./1.0e3)-dq3.*dq6.*t4.*t5.*t6.*t9.*(2.1e1./1.0e3)-dq4.*dq6.*t4.*t5.*t6.*t9.*(2.1e1./1.0e3)+dq3.*dq7.*t4.*t5.*t6.*t10.*(2.1e1./1.0e3)+dq4.*dq7.*t4.*t5.*t6.*t10.*(2.1e1./1.0e3)+dq3.*dq6.*t4.*t7.*t8.*t9.*(2.1e1./1.0e3)+dq4.*dq6.*t4.*t7.*t8.*t9.*(2.1e1./1.0e3)-dq3.*dq7.*t4.*t7.*t8.*t10.*(2.1e1./1.0e3)-dq4.*dq7.*t4.*t7.*t8.*t10.*(2.1e1./1.0e3)+dq5.*dq7.*t5.*t8.*t9.*t10.*(2.1e1./1.0e3)+dq5.*dq7.*t6.*t7.*t9.*t10.*(2.1e1./1.0e3)+dq6.*dq7.*t5.*t6.*t10.*t11.*(2.1e1./1.0e3)-dq6.*dq7.*t7.*t8.*t10.*t11.*(2.1e1./1.0e3)+dq6.*dq7.*t5.*t8.*t9.*t25.*(2.1e1./1.0e3)+dq6.*dq7.*t6.*t7.*t9.*t25.*(2.1e1./1.0e3)-dq5.*dq7.*t4.*t5.*t8.*t10.*t11.*(2.1e1./1.0e3)-dq5.*dq7.*t4.*t6.*t7.*t10.*t11.*(2.1e1./1.0e3)+dq3.*dq7.*t5.*t6.*t9.*t10.*t11.*(2.1e1./1.0e3)+dq4.*dq7.*t5.*t6.*t9.*t10.*t11.*(2.1e1./1.0e3)-dq3.*dq7.*t7.*t8.*t9.*t10.*t11.*(2.1e1./1.0e3)-dq4.*dq7.*t7.*t8.*t9.*t10.*t11.*(2.1e1./1.0e3),t190,t190,-t8.*(-t6.*(dq2.*dq3.*t5.*(2.1e1./1.0e3)+dq2.*dq4.*t5.*(2.1e1./1.0e3))+t8.*(dq2.*dq3.*t7.*(2.1e1./1.0e3)+dq2.*dq4.*t7.*(2.1e1./1.0e3))+dq2.*dq5.*t6.*t139.*(2.1e1./1.0e1))-t10.*(dq7.*t11.*(dq6+t196-dq2.*t4.*t138).*(2.1e1./1.0e3)+dq7.*t10.*(t10.*t194-t11.*t195).*(2.1e1./1.0e3))-dq7.*t153.*(t201+t11.*t194).*1.05e-2+dq6.*t4.*(t196-dq2.*t4.*t138).*(2.1e1./1.0e3)+dq2.*dq5.*t139.*t151.*(2.1e1./2.0e1),t4.*(t211+dq6.*t9.*t200.*(2.1e1./1.0e1)-t9.*t202.*t205)-t9.*(t212+t213+dq6.*t4.*t200.*(2.1e1./1.0e1))+dq7.*t11.*t210.*(2.1e1./1.0e3),t10.*(dq7.*t11.*t210.*(-2.1e1./1.0e1)+t4.*t202.*t205+dq2.*dq5.*t9.*t138.*(2.1e1./1.0e3))-t11.*(t11.*(t212+t213+dq6.*t208.*(2.1e1./1.0e3))+t10.*(t211+dq6.*t195.*(2.1e1./1.0e3)-t9.*t202.*t205)-dq7.*t10.*t210.*(2.1e1./1.0e1))];
end
if nargout > 4
    G = [0.0,0.0,g.*t5.*(-4.3309791)-g.*t7.*5.866623e-2-g.*t5.*t6.*2.136096e-1+g.*t5.*t8.*1.27482732+g.*t6.*t7.*1.27482732+g.*t7.*t8.*2.136096e-1+g.*t4.*t5.*t6.*1.612305e-2-g.*t4.*t7.*t8.*1.612305e-2-g.*t5.*t6.*t9.*4.1238e-4+g.*t5.*t8.*t10.*1.279539e-2+g.*t6.*t7.*t10.*1.279539e-2+g.*t7.*t8.*t9.*4.1238e-4+g.*t5.*t6.*t9.*t11.*1.279539e-2-g.*t7.*t8.*t9.*t11.*1.279539e-2,g.*(t5.*t6.*-2.37344e6+t5.*t8.*1.4164748e7+t6.*t7.*1.4164748e7+t7.*t8.*2.37344e6+t4.*t5.*t6.*1.79145e5-t4.*t7.*t8.*1.79145e5-t5.*t6.*t9.*4.582e3+t5.*t8.*t10.*1.42171e5+t6.*t7.*t10.*1.42171e5+t7.*t8.*t9.*4.582e3+t5.*t6.*t9.*t11.*1.42171e5-t7.*t8.*t9.*t11.*1.42171e5).*9.0e-8,g.*t138.*(t4.*4.582e3+t9.*1.79145e5-t4.*t11.*1.42171e5).*9.0e-8,g.*(t5.*t6.*t11.*1.42171e5-t7.*t8.*t11.*1.42171e5+t5.*t8.*t9.*t10.*1.42171e5+t6.*t7.*t9.*t10.*1.42171e5).*9.0e-8,0.0];
end
